simulink model "model_compatible"  (Simulink 8.7)
(part 8 of 11)

  _CN_29344008_220000_CN_25306938_220000 : powerlib/Elements/Distributed Parameters Line  Phases=3  Frequency=50  Resistance=[0.01273 0.3864]  Inductance="[0.9337e-3  4.1264e-3]"  Capacitance=[12.74e-9 7.751e-9]  Length=40.0884  x1=[8.73114913702011e-11 380000 380000;314.159265358979 314.159265358979 314.159265358979;-0.177670123217348 0.415246442777429 -1.15554988401747]  x2=[1.26090477118469e-09 381852.398472139 381852.398472139;314.159265358979 314.159265358979 314.159265358979;-1.41941675517191 0.415007521738739 -1.15578880505616]  x3=[1.07663708898761e-11 1405.24743813465 1405.24743813466;314.159265358979 314.159265358979 314.159265358979;-2.70558821102223 0.316110507002444 -1.25468581979246]  x4=[8.62234243168895e-12 1405.96374414071 1405.9637441407;314.159265358979 314.159265358979 314.159265358979;0.245769282942371 0.405640215255436 -1.16515611153945]  x5=0.000565541566995742  V1=ones(3,3)  V2=ones(3,3)  I1=ones(3,3)  I2=ones(3,3)  nHarmo=1  Measurements=None
  _CN_29344008_220000_CN_28008024_220000 : powerlib/Elements/Distributed Parameters Line  Phases=3  Frequency=50  Resistance=[0.01273 0.3864]  Inductance="[0.9337e-3  4.1264e-3]"  Capacitance=[12.74e-9 7.751e-9]  Length=70.9833  x1=[8.73114913702011e-11 380000 380000;314.159265358979 314.159265358979 314.159265358979;-0.177670123217348 0.415246442777429 -1.15554988401747]  x2=[1.26090477118469e-09 381852.398472139 381852.398472139;314.159265358979 314.159265358979 314.159265358979;-1.41941675517191 0.415007521738739 -1.15578880505616]  x3=[1.07663708898761e-11 1405.24743813465 1405.24743813466;314.159265358979 314.159265358979 314.159265358979;-2.70558821102223 0.316110507002444 -1.25468581979246]  x4=[8.62234243168895e-12 1405.96374414071 1405.9637441407;314.159265358979 314.159265358979 314.159265358979;0.245769282942371 0.405640215255436 -1.16515611153945]  x5=0.000565541566995742  V1=ones(3,3)  V2=ones(3,3)  I1=ones(3,3)  I2=ones(3,3)  nHarmo=1  Measurements=None
  _CN_29344008_220000_CN_33017336_220000 : powerlib/Elements/Distributed Parameters Line  Phases=3  Frequency=50  Resistance=[0.01273 0.3864]  Inductance="[0.9337e-3  4.1264e-3]"  Capacitance=[12.74e-9 7.751e-9]  Length=11.7304  x1=[8.73114913702011e-11 380000 380000;314.159265358979 314.159265358979 314.159265358979;-0.177670123217348 0.415246442777429 -1.15554988401747]  x2=[1.26090477118469e-09 381852.398472139 381852.398472139;314.159265358979 314.159265358979 314.159265358979;-1.41941675517191 0.415007521738739 -1.15578880505616]  x3=[1.07663708898761e-11 1405.24743813465 1405.24743813466;314.159265358979 314.159265358979 314.159265358979;-2.70558821102223 0.316110507002444 -1.25468581979246]  x4=[8.62234243168895e-12 1405.96374414071 1405.9637441407;314.159265358979 314.159265358979 314.159265358979;0.245769282942371 0.405640215255436 -1.16515611153945]  x5=0.000565541566995742  V1=ones(3,3)  V2=ones(3,3)  I1=ones(3,3)  I2=ones(3,3)  nHarmo=1  Measurements=None
  _CN_29472852_220000_CN_114319248_220000 : powerlib/Elements/Distributed Parameters Line  Phases=3  Frequency=50  Resistance=[0.01273 0.3864]  Inductance="[0.9337e-3  4.1264e-3]"  Capacitance=[12.74e-9 7.751e-9]  Length=21.4615  x1=[8.73114913702011e-11 380000 380000;314.159265358979 314.159265358979 314.159265358979;-0.177670123217348 0.415246442777429 -1.15554988401747]  x2=[1.26090477118469e-09 381852.398472139 381852.398472139;314.159265358979 314.159265358979 314.159265358979;-1.41941675517191 0.415007521738739 -1.15578880505616]  x3=[1.07663708898761e-11 1405.24743813465 1405.24743813466;314.159265358979 314.159265358979 314.159265358979;-2.70558821102223 0.316110507002444 -1.25468581979246]  x4=[8.62234243168895e-12 1405.96374414071 1405.9637441407;314.159265358979 314.159265358979 314.159265358979;0.245769282942371 0.405640215255436 -1.16515611153945]  x5=0.000565541566995742  V1=ones(3,3)  V2=ones(3,3)  I1=ones(3,3)  I2=ones(3,3)  nHarmo=1  Measurements=None
  _CN_29472852_220000_CN_37764852_220000 : powerlib/Elements/Distributed Parameters Line  Phases=3  Frequency=50  Resistance=[0.01273 0.3864]  Inductance="[0.9337e-3  4.1264e-3]"  Capacitance=[12.74e-9 7.751e-9]  Length=46.7716  x1=[8.73114913702011e-11 380000 380000;314.159265358979 314.159265358979 314.159265358979;-0.177670123217348 0.415246442777429 -1.15554988401747]  x2=[1.26090477118469e-09 381852.398472139 381852.398472139;314.159265358979 314.159265358979 314.159265358979;-1.41941675517191 0.415007521738739 -1.15578880505616]  x3=[1.07663708898761e-11 1405.24743813465 1405.24743813466;314.159265358979 314.159265358979 314.159265358979;-2.70558821102223 0.316110507002444 -1.25468581979246]  x4=[8.62234243168895e-12 1405.96374414071 1405.9637441407;314.159265358979 314.159265358979 314.159265358979;0.245769282942371 0.405640215255436 -1.16515611153945]  x5=0.000565541566995742  V1=ones(3,3)  V2=ones(3,3)  I1=ones(3,3)  I2=ones(3,3)  nHarmo=1  Measurements=None
  _CN_29713902_380000_CN218161891 : powerlib/Elements/Distributed Parameters Line  Phases=3  Frequency=50  Resistance=[0.01273 0.3864]  Inductance="[0.9337e-3  4.1264e-3]"  Capacitance=[12.74e-9 7.751e-9]  Length=8.2062  x1=[8.73114913702011e-11 380000 380000;314.159265358979 314.159265358979 314.159265358979;-0.177670123217348 0.415246442777429 -1.15554988401747]  x2=[1.26090477118469e-09 381852.398472139 381852.398472139;314.159265358979 314.159265358979 314.159265358979;-1.41941675517191 0.415007521738739 -1.15578880505616]  x3=[1.07663708898761e-11 1405.24743813465 1405.24743813466;314.159265358979 314.159265358979 314.159265358979;-2.70558821102223 0.316110507002444 -1.25468581979246]  x4=[8.62234243168895e-12 1405.96374414071 1405.9637441407;314.159265358979 314.159265358979 314.159265358979;0.245769282942371 0.405640215255436 -1.16515611153945]  x5=0.000565541566995742  V1=ones(3,3)  V2=ones(3,3)  I1=ones(3,3)  I2=ones(3,3)  nHarmo=1  Measurements=None
  _CN_30132758_380000_CN_43163132_380000 : powerlib/Elements/Distributed Parameters Line  Phases=3  Frequency=50  Resistance=[0.01273 0.3864]  Inductance="[0.9337e-3  4.1264e-3]"  Capacitance=[12.74e-9 7.751e-9]  Length=12.8168  x1=[8.73114913702011e-11 380000 380000;314.159265358979 314.159265358979 314.159265358979;-0.177670123217348 0.415246442777429 -1.15554988401747]  x2=[1.26090477118469e-09 381852.398472139 381852.398472139;314.159265358979 314.159265358979 314.159265358979;-1.41941675517191 0.415007521738739 -1.15578880505616]  x3=[1.07663708898761e-11 1405.24743813465 1405.24743813466;314.159265358979 314.159265358979 314.159265358979;-2.70558821102223 0.316110507002444 -1.25468581979246]  x4=[8.62234243168895e-12 1405.96374414071 1405.9637441407;314.159265358979 314.159265358979 314.159265358979;0.245769282942371 0.405640215255436 -1.16515611153945]  x5=0.000565541566995742  V1=ones(3,3)  V2=ones(3,3)  I1=ones(3,3)  I2=ones(3,3)  nHarmo=1  Measurements=None
  _CN_30164703_380000_CN58421134 : powerlib/Elements/Distributed Parameters Line  Phases=3  Frequency=50  Resistance=[0.01273 0.3864]  Inductance="[0.9337e-3  4.1264e-3]"  Capacitance=[12.74e-9 7.751e-9]  Length=15.2286  x1=[8.73114913702011e-11 380000 380000;314.159265358979 314.159265358979 314.159265358979;-0.177670123217348 0.415246442777429 -1.15554988401747]  x2=[1.26090477118469e-09 381852.398472139 381852.398472139;314.159265358979 314.159265358979 314.159265358979;-1.41941675517191 0.415007521738739 -1.15578880505616]  x3=[1.07663708898761e-11 1405.24743813465 1405.24743813466;314.159265358979 314.159265358979 314.159265358979;-2.70558821102223 0.316110507002444 -1.25468581979246]  x4=[8.62234243168895e-12 1405.96374414071 1405.9637441407;314.159265358979 314.159265358979 314.159265358979;0.245769282942371 0.405640215255436 -1.16515611153945]  x5=0.000565541566995742  V1=ones(3,3)  V2=ones(3,3)  I1=ones(3,3)  I2=ones(3,3)  nHarmo=1  Measurements=None
  _CN_30613895_220000_CN_31019937_220000 : powerlib/Elements/Distributed Parameters Line  Phases=3  Frequency=50  Resistance=[0.01273 0.3864]  Inductance="[0.9337e-3  4.1264e-3]"  Capacitance=[12.74e-9 7.751e-9]  Length=89.562  x1=[8.73114913702011e-11 380000 380000;314.159265358979 314.159265358979 314.159265358979;-0.177670123217348 0.415246442777429 -1.15554988401747]  x2=[1.26090477118469e-09 381852.398472139 381852.398472139;314.159265358979 314.159265358979 314.159265358979;-1.41941675517191 0.415007521738739 -1.15578880505616]  x3=[1.07663708898761e-11 1405.24743813465 1405.24743813466;314.159265358979 314.159265358979 314.159265358979;-2.70558821102223 0.316110507002444 -1.25468581979246]  x4=[8.62234243168895e-12 1405.96374414071 1405.9637441407;314.159265358979 314.159265358979 314.159265358979;0.245769282942371 0.405640215255436 -1.16515611153945]  x5=0.000565541566995742  V1=ones(3,3)  V2=ones(3,3)  I1=ones(3,3)  I2=ones(3,3)  nHarmo=1  Measurements=None
  _CN_30613895_380000_CN_24652261_380000 : powerlib/Elements/Distributed Parameters Line  Phases=3  Frequency=50  Resistance=[0.01273 0.3864]  Inductance="[0.9337e-3  4.1264e-3]"  Capacitance=[12.74e-9 7.751e-9]  Length=77.7493  x1=[8.73114913702011e-11 380000 380000;314.159265358979 314.159265358979 314.159265358979;-0.177670123217348 0.415246442777429 -1.15554988401747]  x2=[1.26090477118469e-09 381852.398472139 381852.398472139;314.159265358979 314.159265358979 314.159265358979;-1.41941675517191 0.415007521738739 -1.15578880505616]  x3=[1.07663708898761e-11 1405.24743813465 1405.24743813466;314.159265358979 314.159265358979 314.159265358979;-2.70558821102223 0.316110507002444 -1.25468581979246]  x4=[8.62234243168895e-12 1405.96374414071 1405.9637441407;314.159265358979 314.159265358979 314.159265358979;0.245769282942371 0.405640215255436 -1.16515611153945]  x5=0.000565541566995742  V1=ones(3,3)  V2=ones(3,3)  I1=ones(3,3)  I2=ones(3,3)  nHarmo=1  Measurements=None
  _CN_30613895_380000_CN_53378027_380000 : powerlib/Elements/Distributed Parameters Line  Phases=3  Frequency=50  Resistance=[0.01273 0.3864]  Inductance="[0.9337e-3  4.1264e-3]"  Capacitance=[12.74e-9 7.751e-9]  Length=52.887  x1=[8.73114913702011e-11 380000 380000;314.159265358979 314.159265358979 314.159265358979;-0.177670123217348 0.415246442777429 -1.15554988401747]  x2=[1.26090477118469e-09 381852.398472139 381852.398472139;314.159265358979 314.159265358979 314.159265358979;-1.41941675517191 0.415007521738739 -1.15578880505616]  x3=[1.07663708898761e-11 1405.24743813465 1405.24743813466;314.159265358979 314.159265358979 314.159265358979;-2.70558821102223 0.316110507002444 -1.25468581979246]  x4=[8.62234243168895e-12 1405.96374414071 1405.9637441407;314.159265358979 314.159265358979 314.159265358979;0.245769282942371 0.405640215255436 -1.16515611153945]  x5=0.000565541566995742  V1=ones(3,3)  V2=ones(3,3)  I1=ones(3,3)  I2=ones(3,3)  nHarmo=1  Measurements=None
  _CN_30622610_220000_CN55015415 : powerlib/Elements/Distributed Parameters Line  Phases=3  Frequency=50  Resistance=[0.01273 0.3864]  Inductance="[0.9337e-3  4.1264e-3]"  Capacitance=[12.74e-9 7.751e-9]  Length=30.8042  x1=[8.73114913702011e-11 380000 380000;314.159265358979 314.159265358979 314.159265358979;-0.177670123217348 0.415246442777429 -1.15554988401747]  x2=[1.26090477118469e-09 381852.398472139 381852.398472139;314.159265358979 314.159265358979 314.159265358979;-1.41941675517191 0.415007521738739 -1.15578880505616]  x3=[1.07663708898761e-11 1405.24743813465 1405.24743813466;314.159265358979 314.159265358979 314.159265358979;-2.70558821102223 0.316110507002444 -1.25468581979246]  x4=[8.62234243168895e-12 1405.96374414071 1405.9637441407;314.159265358979 314.159265358979 314.159265358979;0.245769282942371 0.405640215255436 -1.16515611153945]  x5=0.000565541566995742  V1=ones(3,3)  V2=ones(3,3)  I1=ones(3,3)  I2=ones(3,3)  nHarmo=1  Measurements=None
  _CN_31019937_380000_CN_85523877_380000 : powerlib/Elements/Distributed Parameters Line  Phases=3  Frequency=50  Resistance=[0.01273 0.3864]  Inductance="[0.9337e-3  4.1264e-3]"  Capacitance=[12.74e-9 7.751e-9]  Length=0.24167  x1=[8.73114913702011e-11 380000 380000;314.159265358979 314.159265358979 314.159265358979;-0.177670123217348 0.415246442777429 -1.15554988401747]  x2=[1.26090477118469e-09 381852.398472139 381852.398472139;314.159265358979 314.159265358979 314.159265358979;-1.41941675517191 0.415007521738739 -1.15578880505616]  x3=[1.07663708898761e-11 1405.24743813465 1405.24743813466;314.159265358979 314.159265358979 314.159265358979;-2.70558821102223 0.316110507002444 -1.25468581979246]  x4=[8.62234243168895e-12 1405.96374414071 1405.9637441407;314.159265358979 314.159265358979 314.159265358979;0.245769282942371 0.405640215255436 -1.16515611153945]  x5=0.000565541566995742  V1=ones(3,3)  V2=ones(3,3)  I1=ones(3,3)  I2=ones(3,3)  nHarmo=1  Measurements=None
  _CN_31131320_380000_CN_31131325_380000 : powerlib/Elements/Distributed Parameters Line  Phases=3  Frequency=50  Resistance=[0.01273 0.3864]  Inductance="[0.9337e-3  4.1264e-3]"  Capacitance=[12.74e-9 7.751e-9]  Length=27.2208  x1=[8.73114913702011e-11 380000 380000;314.159265358979 314.159265358979 314.159265358979;-0.177670123217348 0.415246442777429 -1.15554988401747]  x2=[1.26090477118469e-09 381852.398472139 381852.398472139;314.159265358979 314.159265358979 314.159265358979;-1.41941675517191 0.415007521738739 -1.15578880505616]  x3=[1.07663708898761e-11 1405.24743813465 1405.24743813466;314.159265358979 314.159265358979 314.159265358979;-2.70558821102223 0.316110507002444 -1.25468581979246]  x4=[8.62234243168895e-12 1405.96374414071 1405.9637441407;314.159265358979 314.159265358979 314.159265358979;0.245769282942371 0.405640215255436 -1.16515611153945]  x5=0.000565541566995742  V1=ones(3,3)  V2=ones(3,3)  I1=ones(3,3)  I2=ones(3,3)  nHarmo=1  Measurements=None
  _CN_31367937_220000_CN_87653464_220000 : powerlib/Elements/Distributed Parameters Line  Phases=3  Frequency=50  Resistance=[0.01273 0.3864]  Inductance="[0.9337e-3  4.1264e-3]"  Capacitance=[12.74e-9 7.751e-9]  Length=100  x1=[8.73114913702011e-11 380000 380000;314.159265358979 314.159265358979 314.159265358979;-0.177670123217348 0.415246442777429 -1.15554988401747]  x2=[1.26090477118469e-09 381852.398472139 381852.398472139;314.159265358979 314.159265358979 314.159265358979;-1.41941675517191 0.415007521738739 -1.15578880505616]  x3=[1.07663708898761e-11 1405.24743813465 1405.24743813466;314.159265358979 314.159265358979 314.159265358979;-2.70558821102223 0.316110507002444 -1.25468581979246]  x4=[8.62234243168895e-12 1405.96374414071 1405.9637441407;314.159265358979 314.159265358979 314.159265358979;0.245769282942371 0.405640215255436 -1.16515611153945]  x5=0.000565541566995742  V1=ones(3,3)  V2=ones(3,3)  I1=ones(3,3)  I2=ones(3,3)  nHarmo=1  Measurements=None
  _CN_32076853_380000_CN_109582315_380000 : powerlib/Elements/Distributed Parameters Line  Phases=3  Frequency=50  Resistance=[0.01273 0.3864]  Inductance="[0.9337e-3  4.1264e-3]"  Capacitance=[12.74e-9 7.751e-9]  Length=0.34614  x1=[8.73114913702011e-11 380000 380000;314.159265358979 314.159265358979 314.159265358979;-0.177670123217348 0.415246442777429 -1.15554988401747]  x2=[1.26090477118469e-09 381852.398472139 381852.398472139;314.159265358979 314.159265358979 314.159265358979;-1.41941675517191 0.415007521738739 -1.15578880505616]  x3=[1.07663708898761e-11 1405.24743813465 1405.24743813466;314.159265358979 314.159265358979 314.159265358979;-2.70558821102223 0.316110507002444 -1.25468581979246]  x4=[8.62234243168895e-12 1405.96374414071 1405.9637441407;314.159265358979 314.159265358979 314.159265358979;0.245769282942371 0.405640215255436 -1.16515611153945]  x5=0.000565541566995742  V1=ones(3,3)  V2=ones(3,3)  I1=ones(3,3)  I2=ones(3,3)  nHarmo=1  Measurements=None
  _CN_32151621_220000_CN_146962222_220000 : powerlib/Elements/Distributed Parameters Line  Phases=3  Frequency=50  Resistance=[0.01273 0.3864]  Inductance="[0.9337e-3  4.1264e-3]"  Capacitance=[12.74e-9 7.751e-9]  Length=72.3935  x1=[8.73114913702011e-11 380000 380000;314.159265358979 314.159265358979 314.159265358979;-0.177670123217348 0.415246442777429 -1.15554988401747]  x2=[1.26090477118469e-09 381852.398472139 381852.398472139;314.159265358979 314.159265358979 314.159265358979;-1.41941675517191 0.415007521738739 -1.15578880505616]  x3=[1.07663708898761e-11 1405.24743813465 1405.24743813466;314.159265358979 314.159265358979 314.159265358979;-2.70558821102223 0.316110507002444 -1.25468581979246]  x4=[8.62234243168895e-12 1405.96374414071 1405.9637441407;314.159265358979 314.159265358979 314.159265358979;0.245769282942371 0.405640215255436 -1.16515611153945]  x5=0.000565541566995742  V1=ones(3,3)  V2=ones(3,3)  I1=ones(3,3)  I2=ones(3,3)  nHarmo=1  Measurements=None
  _CN_32151621_220000_CN_152261133_220000 : powerlib/Elements/Distributed Parameters Line  Phases=3  Frequency=50  Resistance=[0.01273 0.3864]  Inductance="[0.9337e-3  4.1264e-3]"  Capacitance=[12.74e-9 7.751e-9]  Length=30.7373  x1=[8.73114913702011e-11 380000 380000;314.159265358979 314.159265358979 314.159265358979;-0.177670123217348 0.415246442777429 -1.15554988401747]  x2=[1.26090477118469e-09 381852.398472139 381852.398472139;314.159265358979 314.159265358979 314.159265358979;-1.41941675517191 0.415007521738739 -1.15578880505616]  x3=[1.07663708898761e-11 1405.24743813465 1405.24743813466;314.159265358979 314.159265358979 314.159265358979;-2.70558821102223 0.316110507002444 -1.25468581979246]  x4=[8.62234243168895e-12 1405.96374414071 1405.9637441407;314.159265358979 314.159265358979 314.159265358979;0.245769282942371 0.405640215255436 -1.16515611153945]  x5=0.000565541566995742  V1=ones(3,3)  V2=ones(3,3)  I1=ones(3,3)  I2=ones(3,3)  nHarmo=1  Measurements=None
  _CN_32151621_220000_CN_39011884_220000 : powerlib/Elements/Distributed Parameters Line  Phases=3  Frequency=50  Resistance=[0.01273 0.3864]  Inductance="[0.9337e-3  4.1264e-3]"  Capacitance=[12.74e-9 7.751e-9]  Length=33.2187  x1=[8.73114913702011e-11 380000 380000;314.159265358979 314.159265358979 314.159265358979;-0.177670123217348 0.415246442777429 -1.15554988401747]  x2=[1.26090477118469e-09 381852.398472139 381852.398472139;314.159265358979 314.159265358979 314.159265358979;-1.41941675517191 0.415007521738739 -1.15578880505616]  x3=[1.07663708898761e-11 1405.24743813465 1405.24743813466;314.159265358979 314.159265358979 314.159265358979;-2.70558821102223 0.316110507002444 -1.25468581979246]  x4=[8.62234243168895e-12 1405.96374414071 1405.9637441407;314.159265358979 314.159265358979 314.159265358979;0.245769282942371 0.405640215255436 -1.16515611153945]  x5=0.000565541566995742  V1=ones(3,3)  V2=ones(3,3)  I1=ones(3,3)  I2=ones(3,3)  nHarmo=1  Measurements=None
  _CN_32318130_220000_CN_29389718_220000 : powerlib/Elements/Distributed Parameters Line  Phases=3  Frequency=50  Resistance=[0.01273 0.3864]  Inductance="[0.9337e-3  4.1264e-3]"  Capacitance=[12.74e-9 7.751e-9]  Length=12.1297  x1=[8.73114913702011e-11 380000 380000;314.159265358979 314.159265358979 314.159265358979;-0.177670123217348 0.415246442777429 -1.15554988401747]  x2=[1.26090477118469e-09 381852.398472139 381852.398472139;314.159265358979 314.159265358979 314.159265358979;-1.41941675517191 0.415007521738739 -1.15578880505616]  x3=[1.07663708898761e-11 1405.24743813465 1405.24743813466;314.159265358979 314.159265358979 314.159265358979;-2.70558821102223 0.316110507002444 -1.25468581979246]  x4=[8.62234243168895e-12 1405.96374414071 1405.9637441407;314.159265358979 314.159265358979 314.159265358979;0.245769282942371 0.405640215255436 -1.16515611153945]  x5=0.000565541566995742  V1=ones(3,3)  V2=ones(3,3)  I1=ones(3,3)  I2=ones(3,3)  nHarmo=1  Measurements=None
  _CN_32318130_220000_CN_32062544_220000 : powerlib/Elements/Distributed Parameters Line  Phases=3  Frequency=50  Resistance=[0.01273 0.3864]  Inductance="[0.9337e-3  4.1264e-3]"  Capacitance=[12.74e-9 7.751e-9]  Length=70.4994  x1=[8.73114913702011e-11 380000 380000;314.159265358979 314.159265358979 314.159265358979;-0.177670123217348 0.415246442777429 -1.15554988401747]  x2=[1.26090477118469e-09 381852.398472139 381852.398472139;314.159265358979 314.159265358979 314.159265358979;-1.41941675517191 0.415007521738739 -1.15578880505616]  x3=[1.07663708898761e-11 1405.24743813465 1405.24743813466;314.159265358979 314.159265358979 314.159265358979;-2.70558821102223 0.316110507002444 -1.25468581979246]  x4=[8.62234243168895e-12 1405.96374414071 1405.9637441407;314.159265358979 314.159265358979 314.159265358979;0.245769282942371 0.405640215255436 -1.16515611153945]  x5=0.000565541566995742  V1=ones(3,3)  V2=ones(3,3)  I1=ones(3,3)  I2=ones(3,3)  nHarmo=1  Measurements=None
  _CN_32725957_220000_CN_32725958_220000 : powerlib/Elements/Distributed Parameters Line  Phases=3  Frequency=50  Resistance=[0.01273 0.3864]  Inductance="[0.9337e-3  4.1264e-3]"  Capacitance=[12.74e-9 7.751e-9]  Length=4.0892  x1=[8.73114913702011e-11 380000 380000;314.159265358979 314.159265358979 314.159265358979;-0.177670123217348 0.415246442777429 -1.15554988401747]  x2=[1.26090477118469e-09 381852.398472139 381852.398472139;314.159265358979 314.159265358979 314.159265358979;-1.41941675517191 0.415007521738739 -1.15578880505616]  x3=[1.07663708898761e-11 1405.24743813465 1405.24743813466;314.159265358979 314.159265358979 314.159265358979;-2.70558821102223 0.316110507002444 -1.25468581979246]  x4=[8.62234243168895e-12 1405.96374414071 1405.9637441407;314.159265358979 314.159265358979 314.159265358979;0.245769282942371 0.405640215255436 -1.16515611153945]  x5=0.000565541566995742  V1=ones(3,3)  V2=ones(3,3)  I1=ones(3,3)  I2=ones(3,3)  nHarmo=1  Measurements=None
  _CN_33042984_220000_CN_160093341_220000 : powerlib/Elements/Distributed Parameters Line  Phases=3  Frequency=50  Resistance=[0.01273 0.3864]  Inductance="[0.9337e-3  4.1264e-3]"  Capacitance=[12.74e-9 7.751e-9]  Length=107.68  x1=[8.73114913702011e-11 380000 380000;314.159265358979 314.159265358979 314.159265358979;-0.177670123217348 0.415246442777429 -1.15554988401747]  x2=[1.26090477118469e-09 381852.398472139 381852.398472139;314.159265358979 314.159265358979 314.159265358979;-1.41941675517191 0.415007521738739 -1.15578880505616]  x3=[1.07663708898761e-11 1405.24743813465 1405.24743813466;314.159265358979 314.159265358979 314.159265358979;-2.70558821102223 0.316110507002444 -1.25468581979246]  x4=[8.62234243168895e-12 1405.96374414071 1405.9637441407;314.159265358979 314.159265358979 314.159265358979;0.245769282942371 0.405640215255436 -1.16515611153945]  x5=0.000565541566995742  V1=ones(3,3)  V2=ones(3,3)  I1=ones(3,3)  I2=ones(3,3)  nHarmo=1  Measurements=None
  _CN_33042984_220000_CN_30109913_220000 : powerlib/Elements/Distributed Parameters Line  Phases=3  Frequency=50  Resistance=[0.01273 0.3864]  Inductance="[0.9337e-3  4.1264e-3]"  Capacitance=[12.74e-9 7.751e-9]  Length=79.2206  x1=[8.73114913702011e-11 380000 380000;314.159265358979 314.159265358979 314.159265358979;-0.177670123217348 0.415246442777429 -1.15554988401747]  x2=[1.26090477118469e-09 381852.398472139 381852.398472139;314.159265358979 314.159265358979 314.159265358979;-1.41941675517191 0.415007521738739 -1.15578880505616]  x3=[1.07663708898761e-11 1405.24743813465 1405.24743813466;314.159265358979 314.159265358979 314.159265358979;-2.70558821102223 0.316110507002444 -1.25468581979246]  x4=[8.62234243168895e-12 1405.96374414071 1405.9637441407;314.159265358979 314.159265358979 314.159265358979;0.245769282942371 0.405640215255436 -1.16515611153945]  x5=0.000565541566995742  V1=ones(3,3)  V2=ones(3,3)  I1=ones(3,3)  I2=ones(3,3)  nHarmo=1  Measurements=None
  _CN_33042984_220000_CN_43072656_220000 : powerlib/Elements/Distributed Parameters Line  Phases=3  Frequency=50  Resistance=[0.01273 0.3864]  Inductance="[0.9337e-3  4.1264e-3]"  Capacitance=[12.74e-9 7.751e-9]  Length=148.7412  x1=[8.73114913702011e-11 380000 380000;314.159265358979 314.159265358979 314.159265358979;-0.177670123217348 0.415246442777429 -1.15554988401747]  x2=[1.26090477118469e-09 381852.398472139 381852.398472139;314.159265358979 314.159265358979 314.159265358979;-1.41941675517191 0.415007521738739 -1.15578880505616]  x3=[1.07663708898761e-11 1405.24743813465 1405.24743813466;314.159265358979 314.159265358979 314.159265358979;-2.70558821102223 0.316110507002444 -1.25468581979246]  x4=[8.62234243168895e-12 1405.96374414071 1405.9637441407;314.159265358979 314.159265358979 314.159265358979;0.245769282942371 0.405640215255436 -1.16515611153945]  x5=0.000565541566995742  V1=ones(3,3)  V2=ones(3,3)  I1=ones(3,3)  I2=ones(3,3)  nHarmo=1  Measurements=None
  _CN_33411203_220000_CN_114319248_220000 : powerlib/Elements/Distributed Parameters Line  Phases=3  Frequency=50  Resistance=[0.01273 0.3864]  Inductance="[0.9337e-3  4.1264e-3]"  Capacitance=[12.74e-9 7.751e-9]  Length=100.8638  x1=[8.73114913702011e-11 380000 380000;314.159265358979 314.159265358979 314.159265358979;-0.177670123217348 0.415246442777429 -1.15554988401747]  x2=[1.26090477118469e-09 381852.398472139 381852.398472139;314.159265358979 314.159265358979 314.159265358979;-1.41941675517191 0.415007521738739 -1.15578880505616]  x3=[1.07663708898761e-11 1405.24743813465 1405.24743813466;314.159265358979 314.159265358979 314.159265358979;-2.70558821102223 0.316110507002444 -1.25468581979246]  x4=[8.62234243168895e-12 1405.96374414071 1405.9637441407;314.159265358979 314.159265358979 314.159265358979;0.245769282942371 0.405640215255436 -1.16515611153945]  x5=0.000565541566995742  V1=ones(3,3)  V2=ones(3,3)  I1=ones(3,3)  I2=ones(3,3)  nHarmo=1  Measurements=None
  _CN_33411203_220000_CN_37764852_220000 : powerlib/Elements/Distributed Parameters Line  Phases=3  Frequency=50  Resistance=[0.01273 0.3864]  Inductance="[0.9337e-3  4.1264e-3]"  Capacitance=[12.74e-9 7.751e-9]  Length=34.2315  x1=[8.73114913702011e-11 380000 380000;314.159265358979 314.159265358979 314.159265358979;-0.177670123217348 0.415246442777429 -1.15554988401747]  x2=[1.26090477118469e-09 381852.398472139 381852.398472139;314.159265358979 314.159265358979 314.159265358979;-1.41941675517191 0.415007521738739 -1.15578880505616]  x3=[1.07663708898761e-11 1405.24743813465 1405.24743813466;314.159265358979 314.159265358979 314.159265358979;-2.70558821102223 0.316110507002444 -1.25468581979246]  x4=[8.62234243168895e-12 1405.96374414071 1405.9637441407;314.159265358979 314.159265358979 314.159265358979;0.245769282942371 0.405640215255436 -1.16515611153945]  x5=0.000565541566995742  V1=ones(3,3)  V2=ones(3,3)  I1=ones(3,3)  I2=ones(3,3)  nHarmo=1  Measurements=None
  _CN_33411203_380000_CN_24604789_380000 : powerlib/Elements/Distributed Parameters Line  Phases=3  Frequency=50  Resistance=[0.01273 0.3864]  Inductance="[0.9337e-3  4.1264e-3]"  Capacitance=[12.74e-9 7.751e-9]  Length=143.1283  x1=[8.73114913702011e-11 380000 380000;314.159265358979 314.159265358979 314.159265358979;-0.177670123217348 0.415246442777429 -1.15554988401747]  x2=[1.26090477118469e-09 381852.398472139 381852.398472139;314.159265358979 314.159265358979 314.159265358979;-1.41941675517191 0.415007521738739 -1.15578880505616]  x3=[1.07663708898761e-11 1405.24743813465 1405.24743813466;314.159265358979 314.159265358979 314.159265358979;-2.70558821102223 0.316110507002444 -1.25468581979246]  x4=[8.62234243168895e-12 1405.96374414071 1405.9637441407;314.159265358979 314.159265358979 314.159265358979;0.245769282942371 0.405640215255436 -1.16515611153945]  x5=0.000565541566995742  V1=ones(3,3)  V2=ones(3,3)  I1=ones(3,3)  I2=ones(3,3)  nHarmo=1  Measurements=None
  _CN_33411203_380000_CN_27739871_380000 : powerlib/Elements/Distributed Parameters Line  Phases=3  Frequency=50  Resistance=[0.01273 0.3864]  Inductance="[0.9337e-3  4.1264e-3]"  Capacitance=[12.74e-9 7.751e-9]  Length=129.6976  x1=[8.73114913702011e-11 380000 380000;314.159265358979 314.159265358979 314.159265358979;-0.177670123217348 0.415246442777429 -1.15554988401747]  x2=[1.26090477118469e-09 381852.398472139 381852.398472139;314.159265358979 314.159265358979 314.159265358979;-1.41941675517191 0.415007521738739 -1.15578880505616]  x3=[1.07663708898761e-11 1405.24743813465 1405.24743813466;314.159265358979 314.159265358979 314.159265358979;-2.70558821102223 0.316110507002444 -1.25468581979246]  x4=[8.62234243168895e-12 1405.96374414071 1405.9637441407;314.159265358979 314.159265358979 314.159265358979;0.245769282942371 0.405640215255436 -1.16515611153945]  x5=0.000565541566995742  V1=ones(3,3)  V2=ones(3,3)  I1=ones(3,3)  I2=ones(3,3)  nHarmo=1  Measurements=None
  _CN_35818137_220000_CN_35818522_220000 : powerlib/Elements/Distributed Parameters Line  Phases=3  Frequency=50  Resistance=[0.01273 0.3864]  Inductance="[0.9337e-3  4.1264e-3]"  Capacitance=[12.74e-9 7.751e-9]  Length=1.6839  x1=[8.73114913702011e-11 380000 380000;314.159265358979 314.159265358979 314.159265358979;-0.177670123217348 0.415246442777429 -1.15554988401747]  x2=[1.26090477118469e-09 381852.398472139 381852.398472139;314.159265358979 314.159265358979 314.159265358979;-1.41941675517191 0.415007521738739 -1.15578880505616]  x3=[1.07663708898761e-11 1405.24743813465 1405.24743813466;314.159265358979 314.159265358979 314.159265358979;-2.70558821102223 0.316110507002444 -1.25468581979246]  x4=[8.62234243168895e-12 1405.96374414071 1405.9637441407;314.159265358979 314.159265358979 314.159265358979;0.245769282942371 0.405640215255436 -1.16515611153945]  x5=0.000565541566995742  V1=ones(3,3)  V2=ones(3,3)  I1=ones(3,3)  I2=ones(3,3)  nHarmo=1  Measurements=None
  _CN_35833442_220000_CN125808869 : powerlib/Elements/Distributed Parameters Line  Phases=3  Frequency=50  Resistance=[0.01273 0.3864]  Inductance="[0.9337e-3  4.1264e-3]"  Capacitance=[12.74e-9 7.751e-9]  Length=0.69479  x1=[8.73114913702011e-11 380000 380000;314.159265358979 314.159265358979 314.159265358979;-0.177670123217348 0.415246442777429 -1.15554988401747]  x2=[1.26090477118469e-09 381852.398472139 381852.398472139;314.159265358979 314.159265358979 314.159265358979;-1.41941675517191 0.415007521738739 -1.15578880505616]  x3=[1.07663708898761e-11 1405.24743813465 1405.24743813466;314.159265358979 314.159265358979 314.159265358979;-2.70558821102223 0.316110507002444 -1.25468581979246]  x4=[8.62234243168895e-12 1405.96374414071 1405.9637441407;314.159265358979 314.159265358979 314.159265358979;0.245769282942371 0.405640215255436 -1.16515611153945]  x5=0.000565541566995742  V1=ones(3,3)  V2=ones(3,3)  I1=ones(3,3)  I2=ones(3,3)  nHarmo=1  Measurements=None
  _CN_35833592_220000_CN_35833442_220000 : powerlib/Elements/Distributed Parameters Line  Phases=3  Frequency=50  Resistance=[0.01273 0.3864]  Inductance="[0.9337e-3  4.1264e-3]"  Capacitance=[12.74e-9 7.751e-9]  Length=2.6796  x1=[8.73114913702011e-11 380000 380000;314.159265358979 314.159265358979 314.159265358979;-0.177670123217348 0.415246442777429 -1.15554988401747]  x2=[1.26090477118469e-09 381852.398472139 381852.398472139;314.159265358979 314.159265358979 314.159265358979;-1.41941675517191 0.415007521738739 -1.15578880505616]  x3=[1.07663708898761e-11 1405.24743813465 1405.24743813466;314.159265358979 314.159265358979 314.159265358979;-2.70558821102223 0.316110507002444 -1.25468581979246]  x4=[8.62234243168895e-12 1405.96374414071 1405.9637441407;314.159265358979 314.159265358979 314.159265358979;0.245769282942371 0.405640215255436 -1.16515611153945]  x5=0.000565541566995742  V1=ones(3,3)  V2=ones(3,3)  I1=ones(3,3)  I2=ones(3,3)  nHarmo=1  Measurements=None
  _CN_39690368_220000_CN_32062544_220000 : powerlib/Elements/Distributed Parameters Line  Phases=3  Frequency=50  Resistance=[0.01273 0.3864]  Inductance="[0.9337e-3  4.1264e-3]"  Capacitance=[12.74e-9 7.751e-9]  Length=1.5793  x1=[8.73114913702011e-11 380000 380000;314.159265358979 314.159265358979 314.159265358979;-0.177670123217348 0.415246442777429 -1.15554988401747]  x2=[1.26090477118469e-09 381852.398472139 381852.398472139;314.159265358979 314.159265358979 314.159265358979;-1.41941675517191 0.415007521738739 -1.15578880505616]  x3=[1.07663708898761e-11 1405.24743813465 1405.24743813466;314.159265358979 314.159265358979 314.159265358979;-2.70558821102223 0.316110507002444 -1.25468581979246]  x4=[8.62234243168895e-12 1405.96374414071 1405.9637441407;314.159265358979 314.159265358979 314.159265358979;0.245769282942371 0.405640215255436 -1.16515611153945]  x5=0.000565541566995742  V1=ones(3,3)  V2=ones(3,3)  I1=ones(3,3)  I2=ones(3,3)  nHarmo=1  Measurements=None
  _CN_41334805_220000_CN_143903369_220000 : powerlib/Elements/Distributed Parameters Line  Phases=3  Frequency=50  Resistance=[0.01273 0.3864]  Inductance="[0.9337e-3  4.1264e-3]"  Capacitance=[12.74e-9 7.751e-9]  Length=114.5956  x1=[8.73114913702011e-11 380000 380000;314.159265358979 314.159265358979 314.159265358979;-0.177670123217348 0.415246442777429 -1.15554988401747]  x2=[1.26090477118469e-09 381852.398472139 381852.398472139;314.159265358979 314.159265358979 314.159265358979;-1.41941675517191 0.415007521738739 -1.15578880505616]  x3=[1.07663708898761e-11 1405.24743813465 1405.24743813466;314.159265358979 314.159265358979 314.159265358979;-2.70558821102223 0.316110507002444 -1.25468581979246]  x4=[8.62234243168895e-12 1405.96374414071 1405.9637441407;314.159265358979 314.159265358979 314.159265358979;0.245769282942371 0.405640215255436 -1.16515611153945]  x5=0.000565541566995742  V1=ones(3,3)  V2=ones(3,3)  I1=ones(3,3)  I2=ones(3,3)  nHarmo=1  Measurements=None
  _CN_41334805_220000_CN_152973139_220000 : powerlib/Elements/Distributed Parameters Line  Phases=3  Frequency=50  Resistance=[0.01273 0.3864]  Inductance="[0.9337e-3  4.1264e-3]"  Capacitance=[12.74e-9 7.751e-9]  Length=109.9639  x1=[8.73114913702011e-11 380000 380000;314.159265358979 314.159265358979 314.159265358979;-0.177670123217348 0.415246442777429 -1.15554988401747]  x2=[1.26090477118469e-09 381852.398472139 381852.398472139;314.159265358979 314.159265358979 314.159265358979;-1.41941675517191 0.415007521738739 -1.15578880505616]  x3=[1.07663708898761e-11 1405.24743813465 1405.24743813466;314.159265358979 314.159265358979 314.159265358979;-2.70558821102223 0.316110507002444 -1.25468581979246]  x4=[8.62234243168895e-12 1405.96374414071 1405.9637441407;314.159265358979 314.159265358979 314.159265358979;0.245769282942371 0.405640215255436 -1.16515611153945]  x5=0.000565541566995742  V1=ones(3,3)  V2=ones(3,3)  I1=ones(3,3)  I2=ones(3,3)  nHarmo=1  Measurements=None
  _CN_41334805_220000_CN_207248812_220000 : powerlib/Elements/Distributed Parameters Line  Phases=3  Frequency=50  Resistance=[0.01273 0.3864]  Inductance="[0.9337e-3  4.1264e-3]"  Capacitance=[12.74e-9 7.751e-9]  Length=93.2926  x1=[8.73114913702011e-11 380000 380000;314.159265358979 314.159265358979 314.159265358979;-0.177670123217348 0.415246442777429 -1.15554988401747]  x2=[1.26090477118469e-09 381852.398472139 381852.398472139;314.159265358979 314.159265358979 314.159265358979;-1.41941675517191 0.415007521738739 -1.15578880505616]  x3=[1.07663708898761e-11 1405.24743813465 1405.24743813466;314.159265358979 314.159265358979 314.159265358979;-2.70558821102223 0.316110507002444 -1.25468581979246]  x4=[8.62234243168895e-12 1405.96374414071 1405.9637441407;314.159265358979 314.159265358979 314.159265358979;0.245769282942371 0.405640215255436 -1.16515611153945]  x5=0.000565541566995742  V1=ones(3,3)  V2=ones(3,3)  I1=ones(3,3)  I2=ones(3,3)  nHarmo=1  Measurements=None
  _CN_41334805_220000_CN_23414063_220000 : powerlib/Elements/Distributed Parameters Line  Phases=3  Frequency=50  Resistance=[0.01273 0.3864]  Inductance="[0.9337e-3  4.1264e-3]"  Capacitance=[12.74e-9 7.751e-9]  Length=53.7382  x1=[8.73114913702011e-11 380000 380000;314.159265358979 314.159265358979 314.159265358979;-0.177670123217348 0.415246442777429 -1.15554988401747]  x2=[1.26090477118469e-09 381852.398472139 381852.398472139;314.159265358979 314.159265358979 314.159265358979;-1.41941675517191 0.415007521738739 -1.15578880505616]  x3=[1.07663708898761e-11 1405.24743813465 1405.24743813466;314.159265358979 314.159265358979 314.159265358979;-2.70558821102223 0.316110507002444 -1.25468581979246]  x4=[8.62234243168895e-12 1405.96374414071 1405.9637441407;314.159265358979 314.159265358979 314.159265358979;0.245769282942371 0.405640215255436 -1.16515611153945]  x5=0.000565541566995742  V1=ones(3,3)  V2=ones(3,3)  I1=ones(3,3)  I2=ones(3,3)  nHarmo=1  Measurements=None
  _CN_41334805_220000_CN_25557397_220000 : powerlib/Elements/Distributed Parameters Line  Phases=3  Frequency=50  Resistance=[0.01273 0.3864]  Inductance="[0.9337e-3  4.1264e-3]"  Capacitance=[12.74e-9 7.751e-9]  Length=20.269  x1=[8.73114913702011e-11 380000 380000;314.159265358979 314.159265358979 314.159265358979;-0.177670123217348 0.415246442777429 -1.15554988401747]  x2=[1.26090477118469e-09 381852.398472139 381852.398472139;314.159265358979 314.159265358979 314.159265358979;-1.41941675517191 0.415007521738739 -1.15578880505616]  x3=[1.07663708898761e-11 1405.24743813465 1405.24743813466;314.159265358979 314.159265358979 314.159265358979;-2.70558821102223 0.316110507002444 -1.25468581979246]  x4=[8.62234243168895e-12 1405.96374414071 1405.9637441407;314.159265358979 314.159265358979 314.159265358979;0.245769282942371 0.405640215255436 -1.16515611153945]  x5=0.000565541566995742  V1=ones(3,3)  V2=ones(3,3)  I1=ones(3,3)  I2=ones(3,3)  nHarmo=1  Measurements=None
  _CN_41334805_220000_CN_25786404_220000 : powerlib/Elements/Distributed Parameters Line  Phases=3  Frequency=50  Resistance=[0.01273 0.3864]  Inductance="[0.9337e-3  4.1264e-3]"  Capacitance=[12.74e-9 7.751e-9]  Length=22.5776  x1=[8.73114913702011e-11 380000 380000;314.159265358979 314.159265358979 314.159265358979;-0.177670123217348 0.415246442777429 -1.15554988401747]  x2=[1.26090477118469e-09 381852.398472139 381852.398472139;314.159265358979 314.159265358979 314.159265358979;-1.41941675517191 0.415007521738739 -1.15578880505616]  x3=[1.07663708898761e-11 1405.24743813465 1405.24743813466;314.159265358979 314.159265358979 314.159265358979;-2.70558821102223 0.316110507002444 -1.25468581979246]  x4=[8.62234243168895e-12 1405.96374414071 1405.9637441407;314.159265358979 314.159265358979 314.159265358979;0.245769282942371 0.405640215255436 -1.16515611153945]  x5=0.000565541566995742  V1=ones(3,3)  V2=ones(3,3)  I1=ones(3,3)  I2=ones(3,3)  nHarmo=1  Measurements=None
  _CN_41334805_220000_CN_43688805_220000 : powerlib/Elements/Distributed Parameters Line  Phases=3  Frequency=50  Resistance=[0.01273 0.3864]  Inductance="[0.9337e-3  4.1264e-3]"  Capacitance=[12.74e-9 7.751e-9]  Length=42.9643  x1=[8.73114913702011e-11 380000 380000;314.159265358979 314.159265358979 314.159265358979;-0.177670123217348 0.415246442777429 -1.15554988401747]  x2=[1.26090477118469e-09 381852.398472139 381852.398472139;314.159265358979 314.159265358979 314.159265358979;-1.41941675517191 0.415007521738739 -1.15578880505616]  x3=[1.07663708898761e-11 1405.24743813465 1405.24743813466;314.159265358979 314.159265358979 314.159265358979;-2.70558821102223 0.316110507002444 -1.25468581979246]  x4=[8.62234243168895e-12 1405.96374414071 1405.9637441407;314.159265358979 314.159265358979 314.159265358979;0.245769282942371 0.405640215255436 -1.16515611153945]  x5=0.000565541566995742  V1=ones(3,3)  V2=ones(3,3)  I1=ones(3,3)  I2=ones(3,3)  nHarmo=1  Measurements=None
  _CN_42410916_220000_CN145861680 : powerlib/Elements/Distributed Parameters Line  Phases=3  Frequency=50  Resistance=[0.01273 0.3864]  Inductance="[0.9337e-3  4.1264e-3]"  Capacitance=[12.74e-9 7.751e-9]  Length=1.0748  x1=[8.73114913702011e-11 380000 380000;314.159265358979 314.159265358979 314.159265358979;-0.177670123217348 0.415246442777429 -1.15554988401747]  x2=[1.26090477118469e-09 381852.398472139 381852.398472139;314.159265358979 314.159265358979 314.159265358979;-1.41941675517191 0.415007521738739 -1.15578880505616]  x3=[1.07663708898761e-11 1405.24743813465 1405.24743813466;314.159265358979 314.159265358979 314.159265358979;-2.70558821102223 0.316110507002444 -1.25468581979246]  x4=[8.62234243168895e-12 1405.96374414071 1405.9637441407;314.159265358979 314.159265358979 314.159265358979;0.245769282942371 0.405640215255436 -1.16515611153945]  x5=0.000565541566995742  V1=ones(3,3)  V2=ones(3,3)  I1=ones(3,3)  I2=ones(3,3)  nHarmo=1  Measurements=None
  _CN_42410916_220000_CN_42411962_220000 : powerlib/Elements/Distributed Parameters Line  Phases=3  Frequency=50  Resistance=[0.01273 0.3864]  Inductance="[0.9337e-3  4.1264e-3]"  Capacitance=[12.74e-9 7.751e-9]  Length=0.70686  x1=[8.73114913702011e-11 380000 380000;314.159265358979 314.159265358979 314.159265358979;-0.177670123217348 0.415246442777429 -1.15554988401747]  x2=[1.26090477118469e-09 381852.398472139 381852.398472139;314.159265358979 314.159265358979 314.159265358979;-1.41941675517191 0.415007521738739 -1.15578880505616]  x3=[1.07663708898761e-11 1405.24743813465 1405.24743813466;314.159265358979 314.159265358979 314.159265358979;-2.70558821102223 0.316110507002444 -1.25468581979246]  x4=[8.62234243168895e-12 1405.96374414071 1405.9637441407;314.159265358979 314.159265358979 314.159265358979;0.245769282942371 0.405640215255436 -1.16515611153945]  x5=0.000565541566995742  V1=ones(3,3)  V2=ones(3,3)  I1=ones(3,3)  I2=ones(3,3)  nHarmo=1  Measurements=None
  _CN_42411962_220000_CN145861680 : powerlib/Elements/Distributed Parameters Line  Phases=3  Frequency=50  Resistance=[0.01273 0.3864]  Inductance="[0.9337e-3  4.1264e-3]"  Capacitance=[12.74e-9 7.751e-9]  Length=0.1006  x1=[8.73114913702011e-11 380000 380000;314.159265358979 314.159265358979 314.159265358979;-0.177670123217348 0.415246442777429 -1.15554988401747]  x2=[1.26090477118469e-09 381852.398472139 381852.398472139;314.159265358979 314.159265358979 314.159265358979;-1.41941675517191 0.415007521738739 -1.15578880505616]  x3=[1.07663708898761e-11 1405.24743813465 1405.24743813466;314.159265358979 314.159265358979 314.159265358979;-2.70558821102223 0.316110507002444 -1.25468581979246]  x4=[8.62234243168895e-12 1405.96374414071 1405.9637441407;314.159265358979 314.159265358979 314.159265358979;0.245769282942371 0.405640215255436 -1.16515611153945]  x5=0.000565541566995742  V1=ones(3,3)  V2=ones(3,3)  I1=ones(3,3)  I2=ones(3,3)  nHarmo=1  Measurements=None
  _CN_42488855_380000_CN_112695048_380000 : powerlib/Elements/Distributed Parameters Line  Phases=3  Frequency=50  Resistance=[0.01273 0.3864]  Inductance="[0.9337e-3  4.1264e-3]"  Capacitance=[12.74e-9 7.751e-9]  Length=6.9786  x1=[8.73114913702011e-11 380000 380000;314.159265358979 314.159265358979 314.159265358979;-0.177670123217348 0.415246442777429 -1.15554988401747]  x2=[1.26090477118469e-09 381852.398472139 381852.398472139;314.159265358979 314.159265358979 314.159265358979;-1.41941675517191 0.415007521738739 -1.15578880505616]  x3=[1.07663708898761e-11 1405.24743813465 1405.24743813466;314.159265358979 314.159265358979 314.159265358979;-2.70558821102223 0.316110507002444 -1.25468581979246]  x4=[8.62234243168895e-12 1405.96374414071 1405.9637441407;314.159265358979 314.159265358979 314.159265358979;0.245769282942371 0.405640215255436 -1.16515611153945]  x5=0.000565541566995742  V1=ones(3,3)  V2=ones(3,3)  I1=ones(3,3)  I2=ones(3,3)  nHarmo=1  Measurements=None
  _CN_42488855_380000_CN_22964137_380000 : powerlib/Elements/Distributed Parameters Line  Phases=3  Frequency=50  Resistance=[0.01273 0.3864]  Inductance="[0.9337e-3  4.1264e-3]"  Capacitance=[12.74e-9 7.751e-9]  Length=86.9099  x1=[8.73114913702011e-11 380000 380000;314.159265358979 314.159265358979 314.159265358979;-0.177670123217348 0.415246442777429 -1.15554988401747]  x2=[1.26090477118469e-09 381852.398472139 381852.398472139;314.159265358979 314.159265358979 314.159265358979;-1.41941675517191 0.415007521738739 -1.15578880505616]  x3=[1.07663708898761e-11 1405.24743813465 1405.24743813466;314.159265358979 314.159265358979 314.159265358979;-2.70558821102223 0.316110507002444 -1.25468581979246]  x4=[8.62234243168895e-12 1405.96374414071 1405.9637441407;314.159265358979 314.159265358979 314.159265358979;0.245769282942371 0.405640215255436 -1.16515611153945]  x5=0.000565541566995742  V1=ones(3,3)  V2=ones(3,3)  I1=ones(3,3)  I2=ones(3,3)  nHarmo=1  Measurements=None
  _CN_42488855_380000_CN_32472806_380000 : powerlib/Elements/Distributed Parameters Line  Phases=3  Frequency=50  Resistance=[0.01273 0.3864]  Inductance="[0.9337e-3  4.1264e-3]"  Capacitance=[12.74e-9 7.751e-9]  Length=111.3469  x1=[8.73114913702011e-11 380000 380000;314.159265358979 314.159265358979 314.159265358979;-0.177670123217348 0.415246442777429 -1.15554988401747]  x2=[1.26090477118469e-09 381852.398472139 381852.398472139;314.159265358979 314.159265358979 314.159265358979;-1.41941675517191 0.415007521738739 -1.15578880505616]  x3=[1.07663708898761e-11 1405.24743813465 1405.24743813466;314.159265358979 314.159265358979 314.159265358979;-2.70558821102223 0.316110507002444 -1.25468581979246]  x4=[8.62234243168895e-12 1405.96374414071 1405.9637441407;314.159265358979 314.159265358979 314.159265358979;0.245769282942371 0.405640215255436 -1.16515611153945]  x5=0.000565541566995742  V1=ones(3,3)  V2=ones(3,3)  I1=ones(3,3)  I2=ones(3,3)  nHarmo=1  Measurements=None
  _CN_42488855_380000_CN_35763480_380000 : powerlib/Elements/Distributed Parameters Line  Phases=3  Frequency=50  Resistance=[0.01273 0.3864]  Inductance="[0.9337e-3  4.1264e-3]"  Capacitance=[12.74e-9 7.751e-9]  Length=99.4674  x1=[8.73114913702011e-11 380000 380000;314.159265358979 314.159265358979 314.159265358979;-0.177670123217348 0.415246442777429 -1.15554988401747]  x2=[1.26090477118469e-09 381852.398472139 381852.398472139;314.159265358979 314.159265358979 314.159265358979;-1.41941675517191 0.415007521738739 -1.15578880505616]  x3=[1.07663708898761e-11 1405.24743813465 1405.24743813466;314.159265358979 314.159265358979 314.159265358979;-2.70558821102223 0.316110507002444 -1.25468581979246]  x4=[8.62234243168895e-12 1405.96374414071 1405.9637441407;314.159265358979 314.159265358979 314.159265358979;0.245769282942371 0.405640215255436 -1.16515611153945]  x5=0.000565541566995742  V1=ones(3,3)  V2=ones(3,3)  I1=ones(3,3)  I2=ones(3,3)  nHarmo=1  Measurements=None
  _CN_42488855_380000_CN_42488850_380000 : powerlib/Elements/Distributed Parameters Line  Phases=3  Frequency=50  Resistance=[0.01273 0.3864]  Inductance="[0.9337e-3  4.1264e-3]"  Capacitance=[12.74e-9 7.751e-9]  Length=2.2106  x1=[8.73114913702011e-11 380000 380000;314.159265358979 314.159265358979 314.159265358979;-0.177670123217348 0.415246442777429 -1.15554988401747]  x2=[1.26090477118469e-09 381852.398472139 381852.398472139;314.159265358979 314.159265358979 314.159265358979;-1.41941675517191 0.415007521738739 -1.15578880505616]  x3=[1.07663708898761e-11 1405.24743813465 1405.24743813466;314.159265358979 314.159265358979 314.159265358979;-2.70558821102223 0.316110507002444 -1.25468581979246]  x4=[8.62234243168895e-12 1405.96374414071 1405.9637441407;314.159265358979 314.159265358979 314.159265358979;0.245769282942371 0.405640215255436 -1.16515611153945]  x5=0.000565541566995742  V1=ones(3,3)  V2=ones(3,3)  I1=ones(3,3)  I2=ones(3,3)  nHarmo=1  Measurements=None
  _CN_42488855_380000_CN_42809973_380000 : powerlib/Elements/Distributed Parameters Line  Phases=3  Frequency=50  Resistance=[0.01273 0.3864]  Inductance="[0.9337e-3  4.1264e-3]"  Capacitance=[12.74e-9 7.751e-9]  Length=46.214  x1=[8.73114913702011e-11 380000 380000;314.159265358979 314.159265358979 314.159265358979;-0.177670123217348 0.415246442777429 -1.15554988401747]  x2=[1.26090477118469e-09 381852.398472139 381852.398472139;314.159265358979 314.159265358979 314.159265358979;-1.41941675517191 0.415007521738739 -1.15578880505616]  x3=[1.07663708898761e-11 1405.24743813465 1405.24743813466;314.159265358979 314.159265358979 314.159265358979;-2.70558821102223 0.316110507002444 -1.25468581979246]  x4=[8.62234243168895e-12 1405.96374414071 1405.9637441407;314.159265358979 314.159265358979 314.159265358979;0.245769282942371 0.405640215255436 -1.16515611153945]  x5=0.000565541566995742  V1=ones(3,3)  V2=ones(3,3)  I1=ones(3,3)  I2=ones(3,3)  nHarmo=1  Measurements=None
  _CN_42681484_380000_CN_24413992_380000 : powerlib/Elements/Distributed Parameters Line  Phases=3  Frequency=50  Resistance=[0.01273 0.3864]  Inductance="[0.9337e-3  4.1264e-3]"  Capacitance=[12.74e-9 7.751e-9]  Length=47.1732  x1=[8.73114913702011e-11 380000 380000;314.159265358979 314.159265358979 314.159265358979;-0.177670123217348 0.415246442777429 -1.15554988401747]  x2=[1.26090477118469e-09 381852.398472139 381852.398472139;314.159265358979 314.159265358979 314.159265358979;-1.41941675517191 0.415007521738739 -1.15578880505616]  x3=[1.07663708898761e-11 1405.24743813465 1405.24743813466;314.159265358979 314.159265358979 314.159265358979;-2.70558821102223 0.316110507002444 -1.25468581979246]  x4=[8.62234243168895e-12 1405.96374414071 1405.9637441407;314.159265358979 314.159265358979 314.159265358979;0.245769282942371 0.405640215255436 -1.16515611153945]  x5=0.000565541566995742  V1=ones(3,3)  V2=ones(3,3)  I1=ones(3,3)  I2=ones(3,3)  nHarmo=1  Measurements=None
  _CN_42681484_380000_CN_274630377_380000 : powerlib/Elements/Distributed Parameters Line  Phases=3  Frequency=50  Resistance=[0.01273 0.3864]  Inductance="[0.9337e-3  4.1264e-3]"  Capacitance=[12.74e-9 7.751e-9]  Length=45.3031  x1=[8.73114913702011e-11 380000 380000;314.159265358979 314.159265358979 314.159265358979;-0.177670123217348 0.415246442777429 -1.15554988401747]  x2=[1.26090477118469e-09 381852.398472139 381852.398472139;314.159265358979 314.159265358979 314.159265358979;-1.41941675517191 0.415007521738739 -1.15578880505616]  x3=[1.07663708898761e-11 1405.24743813465 1405.24743813466;314.159265358979 314.159265358979 314.159265358979;-2.70558821102223 0.316110507002444 -1.25468581979246]  x4=[8.62234243168895e-12 1405.96374414071 1405.9637441407;314.159265358979 314.159265358979 314.159265358979;0.245769282942371 0.405640215255436 -1.16515611153945]  x5=0.000565541566995742  V1=ones(3,3)  V2=ones(3,3)  I1=ones(3,3)  I2=ones(3,3)  nHarmo=1  Measurements=None
  _CN_43163132_380000_CN185569568 : powerlib/Elements/Distributed Parameters Line  Phases=3  Frequency=50  Resistance=[0.01273 0.3864]  Inductance="[0.9337e-3  4.1264e-3]"  Capacitance=[12.74e-9 7.751e-9]  Length=2.1561  x1=[8.73114913702011e-11 380000 380000;314.159265358979 314.159265358979 314.159265358979;-0.177670123217348 0.415246442777429 -1.15554988401747]  x2=[1.26090477118469e-09 381852.398472139 381852.398472139;314.159265358979 314.159265358979 314.159265358979;-1.41941675517191 0.415007521738739 -1.15578880505616]  x3=[1.07663708898761e-11 1405.24743813465 1405.24743813466;314.159265358979 314.159265358979 314.159265358979;-2.70558821102223 0.316110507002444 -1.25468581979246]  x4=[8.62234243168895e-12 1405.96374414071 1405.9637441407;314.159265358979 314.159265358979 314.159265358979;0.245769282942371 0.405640215255436 -1.16515611153945]  x5=0.000565541566995742  V1=ones(3,3)  V2=ones(3,3)  I1=ones(3,3)  I2=ones(3,3)  nHarmo=1  Measurements=None
  _CN_46766896_220000_CN_90807341_220000 : powerlib/Elements/Distributed Parameters Line  Phases=3  Frequency=50  Resistance=[0.01273 0.3864]  Inductance="[0.9337e-3  4.1264e-3]"  Capacitance=[12.74e-9 7.751e-9]  Length=0.24571  x1=[8.73114913702011e-11 380000 380000;314.159265358979 314.159265358979 314.159265358979;-0.177670123217348 0.415246442777429 -1.15554988401747]  x2=[1.26090477118469e-09 381852.398472139 381852.398472139;314.159265358979 314.159265358979 314.159265358979;-1.41941675517191 0.415007521738739 -1.15578880505616]  x3=[1.07663708898761e-11 1405.24743813465 1405.24743813466;314.159265358979 314.159265358979 314.159265358979;-2.70558821102223 0.316110507002444 -1.25468581979246]  x4=[8.62234243168895e-12 1405.96374414071 1405.9637441407;314.159265358979 314.159265358979 314.159265358979;0.245769282942371 0.405640215255436 -1.16515611153945]  x5=0.000565541566995742  V1=ones(3,3)  V2=ones(3,3)  I1=ones(3,3)  I2=ones(3,3)  nHarmo=1  Measurements=None
  _CN_54359256_220000_CN30425117 : powerlib/Elements/Distributed Parameters Line  Phases=3  Frequency=50  Resistance=[0.01273 0.3864]  Inductance="[0.9337e-3  4.1264e-3]"  Capacitance=[12.74e-9 7.751e-9]  Length=9.0385  x1=[8.73114913702011e-11 380000 380000;314.159265358979 314.159265358979 314.159265358979;-0.177670123217348 0.415246442777429 -1.15554988401747]  x2=[1.26090477118469e-09 381852.398472139 381852.398472139;314.159265358979 314.159265358979 314.159265358979;-1.41941675517191 0.415007521738739 -1.15578880505616]  x3=[1.07663708898761e-11 1405.24743813465 1405.24743813466;314.159265358979 314.159265358979 314.159265358979;-2.70558821102223 0.316110507002444 -1.25468581979246]  x4=[8.62234243168895e-12 1405.96374414071 1405.9637441407;314.159265358979 314.159265358979 314.159265358979;0.245769282942371 0.405640215255436 -1.16515611153945]  x5=0.000565541566995742  V1=ones(3,3)  V2=ones(3,3)  I1=ones(3,3)  I2=ones(3,3)  nHarmo=1  Measurements=None
  _CN_54359256_220000_CN_100812630_220000 : powerlib/Elements/Distributed Parameters Line  Phases=3  Frequency=50  Resistance=[0.01273 0.3864]  Inductance="[0.9337e-3  4.1264e-3]"  Capacitance=[12.74e-9 7.751e-9]  Length=9.0478  x1=[8.73114913702011e-11 380000 380000;314.159265358979 314.159265358979 314.159265358979;-0.177670123217348 0.415246442777429 -1.15554988401747]  x2=[1.26090477118469e-09 381852.398472139 381852.398472139;314.159265358979 314.159265358979 314.159265358979;-1.41941675517191 0.415007521738739 -1.15578880505616]  x3=[1.07663708898761e-11 1405.24743813465 1405.24743813466;314.159265358979 314.159265358979 314.159265358979;-2.70558821102223 0.316110507002444 -1.25468581979246]  x4=[8.62234243168895e-12 1405.96374414071 1405.9637441407;314.159265358979 314.159265358979 314.159265358979;0.245769282942371 0.405640215255436 -1.16515611153945]  x5=0.000565541566995742  V1=ones(3,3)  V2=ones(3,3)  I1=ones(3,3)  I2=ones(3,3)  nHarmo=1  Measurements=None
  _CN_54359256_380000_CN115145869 : powerlib/Elements/Distributed Parameters Line  Phases=3  Frequency=50  Resistance=[0.01273 0.3864]  Inductance="[0.9337e-3  4.1264e-3]"  Capacitance=[12.74e-9 7.751e-9]  Length=35.9283  x1=[8.73114913702011e-11 380000 380000;314.159265358979 314.159265358979 314.159265358979;-0.177670123217348 0.415246442777429 -1.15554988401747]  x2=[1.26090477118469e-09 381852.398472139 381852.398472139;314.159265358979 314.159265358979 314.159265358979;-1.41941675517191 0.415007521738739 -1.15578880505616]  x3=[1.07663708898761e-11 1405.24743813465 1405.24743813466;314.159265358979 314.159265358979 314.159265358979;-2.70558821102223 0.316110507002444 -1.25468581979246]  x4=[8.62234243168895e-12 1405.96374414071 1405.9637441407;314.159265358979 314.159265358979 314.159265358979;0.245769282942371 0.405640215255436 -1.16515611153945]  x5=0.000565541566995742  V1=ones(3,3)  V2=ones(3,3)  I1=ones(3,3)  I2=ones(3,3)  nHarmo=1  Measurements=None
  _CN_59026005_380000_CN_157807291_380000 : powerlib/Elements/Distributed Parameters Line  Phases=3  Frequency=50  Resistance=[0.01273 0.3864]  Inductance="[0.9337e-3  4.1264e-3]"  Capacitance=[12.74e-9 7.751e-9]  Length=90.2072  x1=[8.73114913702011e-11 380000 380000;314.159265358979 314.159265358979 314.159265358979;-0.177670123217348 0.415246442777429 -1.15554988401747]  x2=[1.26090477118469e-09 381852.398472139 381852.398472139;314.159265358979 314.159265358979 314.159265358979;-1.41941675517191 0.415007521738739 -1.15578880505616]  x3=[1.07663708898761e-11 1405.24743813465 1405.24743813466;314.159265358979 314.159265358979 314.159265358979;-2.70558821102223 0.316110507002444 -1.25468581979246]  x4=[8.62234243168895e-12 1405.96374414071 1405.9637441407;314.159265358979 314.159265358979 314.159265358979;0.245769282942371 0.405640215255436 -1.16515611153945]  x5=0.000565541566995742  V1=ones(3,3)  V2=ones(3,3)  I1=ones(3,3)  I2=ones(3,3)  nHarmo=1  Measurements=None
  _CN_59925390_380000_CN_113546939_380000 : powerlib/Elements/Distributed Parameters Line  Phases=3  Frequency=50  Resistance=[0.01273 0.3864]  Inductance="[0.9337e-3  4.1264e-3]"  Capacitance=[12.74e-9 7.751e-9]  Length=23.5758  x1=[8.73114913702011e-11 380000 380000;314.159265358979 314.159265358979 314.159265358979;-0.177670123217348 0.415246442777429 -1.15554988401747]  x2=[1.26090477118469e-09 381852.398472139 381852.398472139;314.159265358979 314.159265358979 314.159265358979;-1.41941675517191 0.415007521738739 -1.15578880505616]  x3=[1.07663708898761e-11 1405.24743813465 1405.24743813466;314.159265358979 314.159265358979 314.159265358979;-2.70558821102223 0.316110507002444 -1.25468581979246]  x4=[8.62234243168895e-12 1405.96374414071 1405.9637441407;314.159265358979 314.159265358979 314.159265358979;0.245769282942371 0.405640215255436 -1.16515611153945]  x5=0.000565541566995742  V1=ones(3,3)  V2=ones(3,3)  I1=ones(3,3)  I2=ones(3,3)  nHarmo=1  Measurements=None
  _CN_60032354_220000_CN55015415 : powerlib/Elements/Distributed Parameters Line  Phases=3  Frequency=50  Resistance=[0.01273 0.3864]  Inductance="[0.9337e-3  4.1264e-3]"  Capacitance=[12.74e-9 7.751e-9]  Length=0.32568  x1=[8.73114913702011e-11 380000 380000;314.159265358979 314.159265358979 314.159265358979;-0.177670123217348 0.415246442777429 -1.15554988401747]  x2=[1.26090477118469e-09 381852.398472139 381852.398472139;314.159265358979 314.159265358979 314.159265358979;-1.41941675517191 0.415007521738739 -1.15578880505616]  x3=[1.07663708898761e-11 1405.24743813465 1405.24743813466;314.159265358979 314.159265358979 314.159265358979;-2.70558821102223 0.316110507002444 -1.25468581979246]  x4=[8.62234243168895e-12 1405.96374414071 1405.9637441407;314.159265358979 314.159265358979 314.159265358979;0.245769282942371 0.405640215255436 -1.16515611153945]  x5=0.000565541566995742  V1=ones(3,3)  V2=ones(3,3)  I1=ones(3,3)  I2=ones(3,3)  nHarmo=1  Measurements=None
  _CN_61918154_380000_CN49339874 : powerlib/Elements/Distributed Parameters Line  Phases=3  Frequency=50  Resistance=[0.01273 0.3864]  Inductance="[0.9337e-3  4.1264e-3]"  Capacitance=[12.74e-9 7.751e-9]  Length=1.4703  x1=[8.73114913702011e-11 380000 380000;314.159265358979 314.159265358979 314.159265358979;-0.177670123217348 0.415246442777429 -1.15554988401747]  x2=[1.26090477118469e-09 381852.398472139 381852.398472139;314.159265358979 314.159265358979 314.159265358979;-1.41941675517191 0.415007521738739 -1.15578880505616]  x3=[1.07663708898761e-11 1405.24743813465 1405.24743813466;314.159265358979 314.159265358979 314.159265358979;-2.70558821102223 0.316110507002444 -1.25468581979246]  x4=[8.62234243168895e-12 1405.96374414071 1405.9637441407;314.159265358979 314.159265358979 314.159265358979;0.245769282942371 0.405640215255436 -1.16515611153945]  x5=0.000565541566995742  V1=ones(3,3)  V2=ones(3,3)  I1=ones(3,3)  I2=ones(3,3)  nHarmo=1  Measurements=None
  _CN_63114179_380000_CN_35763480_380000 : powerlib/Elements/Distributed Parameters Line  Phases=3  Frequency=50  Resistance=[0.01273 0.3864]  Inductance="[0.9337e-3  4.1264e-3]"  Capacitance=[12.74e-9 7.751e-9]  Length=28.0497  x1=[8.73114913702011e-11 380000 380000;314.159265358979 314.159265358979 314.159265358979;-0.177670123217348 0.415246442777429 -1.15554988401747]  x2=[1.26090477118469e-09 381852.398472139 381852.398472139;314.159265358979 314.159265358979 314.159265358979;-1.41941675517191 0.415007521738739 -1.15578880505616]  x3=[1.07663708898761e-11 1405.24743813465 1405.24743813466;314.159265358979 314.159265358979 314.159265358979;-2.70558821102223 0.316110507002444 -1.25468581979246]  x4=[8.62234243168895e-12 1405.96374414071 1405.9637441407;314.159265358979 314.159265358979 314.159265358979;0.245769282942371 0.405640215255436 -1.16515611153945]  x5=0.000565541566995742  V1=ones(3,3)  V2=ones(3,3)  I1=ones(3,3)  I2=ones(3,3)  nHarmo=1  Measurements=None
  _CN_66038431_220000_CN131986820 : powerlib/Elements/Distributed Parameters Line  Phases=3  Frequency=50  Resistance=[0.01273 0.3864]  Inductance="[0.9337e-3  4.1264e-3]"  Capacitance=[12.74e-9 7.751e-9]  Length=60.8249  x1=[8.73114913702011e-11 380000 380000;314.159265358979 314.159265358979 314.159265358979;-0.177670123217348 0.415246442777429 -1.15554988401747]  x2=[1.26090477118469e-09 381852.398472139 381852.398472139;314.159265358979 314.159265358979 314.159265358979;-1.41941675517191 0.415007521738739 -1.15578880505616]  x3=[1.07663708898761e-11 1405.24743813465 1405.24743813466;314.159265358979 314.159265358979 314.159265358979;-2.70558821102223 0.316110507002444 -1.25468581979246]  x4=[8.62234243168895e-12 1405.96374414071 1405.9637441407;314.159265358979 314.159265358979 314.159265358979;0.245769282942371 0.405640215255436 -1.16515611153945]  x5=0.000565541566995742  V1=ones(3,3)  V2=ones(3,3)  I1=ones(3,3)  I2=ones(3,3)  nHarmo=1  Measurements=None
  _CN_66038431_220000_CN_113546939_220000 : powerlib/Elements/Distributed Parameters Line  Phases=3  Frequency=50  Resistance=[0.01273 0.3864]  Inductance="[0.9337e-3  4.1264e-3]"  Capacitance=[12.74e-9 7.751e-9]  Length=43.3852  x1=[8.73114913702011e-11 380000 380000;314.159265358979 314.159265358979 314.159265358979;-0.177670123217348 0.415246442777429 -1.15554988401747]  x2=[1.26090477118469e-09 381852.398472139 381852.398472139;314.159265358979 314.159265358979 314.159265358979;-1.41941675517191 0.415007521738739 -1.15578880505616]  x3=[1.07663708898761e-11 1405.24743813465 1405.24743813466;314.159265358979 314.159265358979 314.159265358979;-2.70558821102223 0.316110507002444 -1.25468581979246]  x4=[8.62234243168895e-12 1405.96374414071 1405.9637441407;314.159265358979 314.159265358979 314.159265358979;0.245769282942371 0.405640215255436 -1.16515611153945]  x5=0.000565541566995742  V1=ones(3,3)  V2=ones(3,3)  I1=ones(3,3)  I2=ones(3,3)  nHarmo=1  Measurements=None
  _CN_66038431_220000_CN_24667346_220000 : powerlib/Elements/Distributed Parameters Line  Phases=3  Frequency=50  Resistance=[0.01273 0.3864]  Inductance="[0.9337e-3  4.1264e-3]"  Capacitance=[12.74e-9 7.751e-9]  Length=67.0965  x1=[8.73114913702011e-11 380000 380000;314.159265358979 314.159265358979 314.159265358979;-0.177670123217348 0.415246442777429 -1.15554988401747]  x2=[1.26090477118469e-09 381852.398472139 381852.398472139;314.159265358979 314.159265358979 314.159265358979;-1.41941675517191 0.415007521738739 -1.15578880505616]  x3=[1.07663708898761e-11 1405.24743813465 1405.24743813466;314.159265358979 314.159265358979 314.159265358979;-2.70558821102223 0.316110507002444 -1.25468581979246]  x4=[8.62234243168895e-12 1405.96374414071 1405.9637441407;314.159265358979 314.159265358979 314.159265358979;0.245769282942371 0.405640215255436 -1.16515611153945]  x5=0.000565541566995742  V1=ones(3,3)  V2=ones(3,3)  I1=ones(3,3)  I2=ones(3,3)  nHarmo=1  Measurements=None
  _CN_66038431_220000_CN_28452784_220000 : powerlib/Elements/Distributed Parameters Line  Phases=3  Frequency=50  Resistance=[0.01273 0.3864]  Inductance="[0.9337e-3  4.1264e-3]"  Capacitance=[12.74e-9 7.751e-9]  Length=20.5572  x1=[8.73114913702011e-11 380000 380000;314.159265358979 314.159265358979 314.159265358979;-0.177670123217348 0.415246442777429 -1.15554988401747]  x2=[1.26090477118469e-09 381852.398472139 381852.398472139;314.159265358979 314.159265358979 314.159265358979;-1.41941675517191 0.415007521738739 -1.15578880505616]  x3=[1.07663708898761e-11 1405.24743813465 1405.24743813466;314.159265358979 314.159265358979 314.159265358979;-2.70558821102223 0.316110507002444 -1.25468581979246]  x4=[8.62234243168895e-12 1405.96374414071 1405.9637441407;314.159265358979 314.159265358979 314.159265358979;0.245769282942371 0.405640215255436 -1.16515611153945]  x5=0.000565541566995742  V1=ones(3,3)  V2=ones(3,3)  I1=ones(3,3)  I2=ones(3,3)  nHarmo=1  Measurements=None
  _CN_68532663_220000_CN252655527 : powerlib/Elements/Distributed Parameters Line  Phases=3  Frequency=50  Resistance=[0.01273 0.3864]  Inductance="[0.9337e-3  4.1264e-3]"  Capacitance=[12.74e-9 7.751e-9]  Length=0.11054  x1=[8.73114913702011e-11 380000 380000;314.159265358979 314.159265358979 314.159265358979;-0.177670123217348 0.415246442777429 -1.15554988401747]  x2=[1.26090477118469e-09 381852.398472139 381852.398472139;314.159265358979 314.159265358979 314.159265358979;-1.41941675517191 0.415007521738739 -1.15578880505616]  x3=[1.07663708898761e-11 1405.24743813465 1405.24743813466;314.159265358979 314.159265358979 314.159265358979;-2.70558821102223 0.316110507002444 -1.25468581979246]  x4=[8.62234243168895e-12 1405.96374414071 1405.9637441407;314.159265358979 314.159265358979 314.159265358979;0.245769282942371 0.405640215255436 -1.16515611153945]  x5=0.000565541566995742  V1=ones(3,3)  V2=ones(3,3)  I1=ones(3,3)  I2=ones(3,3)  nHarmo=1  Measurements=None
  _CN_68532663_220000_CN_24237879_220000 : powerlib/Elements/Distributed Parameters Line  Phases=3  Frequency=50  Resistance=[0.01273 0.3864]  Inductance="[0.9337e-3  4.1264e-3]"  Capacitance=[12.74e-9 7.751e-9]  Length=107.5033  x1=[8.73114913702011e-11 380000 380000;314.159265358979 314.159265358979 314.159265358979;-0.177670123217348 0.415246442777429 -1.15554988401747]  x2=[1.26090477118469e-09 381852.398472139 381852.398472139;314.159265358979 314.159265358979 314.159265358979;-1.41941675517191 0.415007521738739 -1.15578880505616]  x3=[1.07663708898761e-11 1405.24743813465 1405.24743813466;314.159265358979 314.159265358979 314.159265358979;-2.70558821102223 0.316110507002444 -1.25468581979246]  x4=[8.62234243168895e-12 1405.96374414071 1405.9637441407;314.159265358979 314.159265358979 314.159265358979;0.245769282942371 0.405640215255436 -1.16515611153945]  x5=0.000565541566995742  V1=ones(3,3)  V2=ones(3,3)  I1=ones(3,3)  I2=ones(3,3)  nHarmo=1  Measurements=None
  _CN_74893659_380000_CN_74893662_380000 : powerlib/Elements/Distributed Parameters Line  Phases=3  Frequency=50  Resistance=[0.01273 0.3864]  Inductance="[0.9337e-3  4.1264e-3]"  Capacitance=[12.74e-9 7.751e-9]  Length=5.071  x1=[8.73114913702011e-11 380000 380000;314.159265358979 314.159265358979 314.159265358979;-0.177670123217348 0.415246442777429 -1.15554988401747]  x2=[1.26090477118469e-09 381852.398472139 381852.398472139;314.159265358979 314.159265358979 314.159265358979;-1.41941675517191 0.415007521738739 -1.15578880505616]  x3=[1.07663708898761e-11 1405.24743813465 1405.24743813466;314.159265358979 314.159265358979 314.159265358979;-2.70558821102223 0.316110507002444 -1.25468581979246]  x4=[8.62234243168895e-12 1405.96374414071 1405.9637441407;314.159265358979 314.159265358979 314.159265358979;0.245769282942371 0.405640215255436 -1.16515611153945]  x5=0.000565541566995742  V1=ones(3,3)  V2=ones(3,3)  I1=ones(3,3)  I2=ones(3,3)  nHarmo=1  Measurements=None
  _CN_76185022_380000_CN26623135 : powerlib/Elements/Distributed Parameters Line  Phases=3  Frequency=50  Resistance=[0.01273 0.3864]  Inductance="[0.9337e-3  4.1264e-3]"  Capacitance=[12.74e-9 7.751e-9]  Length=9.9331  x1=[8.73114913702011e-11 380000 380000;314.159265358979 314.159265358979 314.159265358979;-0.177670123217348 0.415246442777429 -1.15554988401747]  x2=[1.26090477118469e-09 381852.398472139 381852.398472139;314.159265358979 314.159265358979 314.159265358979;-1.41941675517191 0.415007521738739 -1.15578880505616]  x3=[1.07663708898761e-11 1405.24743813465 1405.24743813466;314.159265358979 314.159265358979 314.159265358979;-2.70558821102223 0.316110507002444 -1.25468581979246]  x4=[8.62234243168895e-12 1405.96374414071 1405.9637441407;314.159265358979 314.159265358979 314.159265358979;0.245769282942371 0.405640215255436 -1.16515611153945]  x5=0.000565541566995742  V1=ones(3,3)  V2=ones(3,3)  I1=ones(3,3)  I2=ones(3,3)  nHarmo=1  Measurements=None
  _CN_77697810_380000_CN23802422 : powerlib/Elements/Distributed Parameters Line  Phases=3  Frequency=50  Resistance=[0.01273 0.3864]  Inductance="[0.9337e-3  4.1264e-3]"  Capacitance=[12.74e-9 7.751e-9]  Length=0.29708  x1=[8.73114913702011e-11 380000 380000;314.159265358979 314.159265358979 314.159265358979;-0.177670123217348 0.415246442777429 -1.15554988401747]  x2=[1.26090477118469e-09 381852.398472139 381852.398472139;314.159265358979 314.159265358979 314.159265358979;-1.41941675517191 0.415007521738739 -1.15578880505616]  x3=[1.07663708898761e-11 1405.24743813465 1405.24743813466;314.159265358979 314.159265358979 314.159265358979;-2.70558821102223 0.316110507002444 -1.25468581979246]  x4=[8.62234243168895e-12 1405.96374414071 1405.9637441407;314.159265358979 314.159265358979 314.159265358979;0.245769282942371 0.405640215255436 -1.16515611153945]  x5=0.000565541566995742  V1=ones(3,3)  V2=ones(3,3)  I1=ones(3,3)  I2=ones(3,3)  nHarmo=1  Measurements=None
  _CN_77697810_380000_CN_24976300_380000 : powerlib/Elements/Distributed Parameters Line  Phases=3  Frequency=50  Resistance=[0.01273 0.3864]  Inductance="[0.9337e-3  4.1264e-3]"  Capacitance=[12.74e-9 7.751e-9]  Length=96.0007  x1=[8.73114913702011e-11 380000 380000;314.159265358979 314.159265358979 314.159265358979;-0.177670123217348 0.415246442777429 -1.15554988401747]  x2=[1.26090477118469e-09 381852.398472139 381852.398472139;314.159265358979 314.159265358979 314.159265358979;-1.41941675517191 0.415007521738739 -1.15578880505616]  x3=[1.07663708898761e-11 1405.24743813465 1405.24743813466;314.159265358979 314.159265358979 314.159265358979;-2.70558821102223 0.316110507002444 -1.25468581979246]  x4=[8.62234243168895e-12 1405.96374414071 1405.9637441407;314.159265358979 314.159265358979 314.159265358979;0.245769282942371 0.405640215255436 -1.16515611153945]  x5=0.000565541566995742  V1=ones(3,3)  V2=ones(3,3)  I1=ones(3,3)  I2=ones(3,3)  nHarmo=1  Measurements=None
  _CN_82310607_220000_CN_90109304_220000 : powerlib/Elements/Distributed Parameters Line  Phases=3  Frequency=50  Resistance=[0.01273 0.3864]  Inductance="[0.9337e-3  4.1264e-3]"  Capacitance=[12.74e-9 7.751e-9]  Length=1.995  x1=[8.73114913702011e-11 380000 380000;314.159265358979 314.159265358979 314.159265358979;-0.177670123217348 0.415246442777429 -1.15554988401747]  x2=[1.26090477118469e-09 381852.398472139 381852.398472139;314.159265358979 314.159265358979 314.159265358979;-1.41941675517191 0.415007521738739 -1.15578880505616]  x3=[1.07663708898761e-11 1405.24743813465 1405.24743813466;314.159265358979 314.159265358979 314.159265358979;-2.70558821102223 0.316110507002444 -1.25468581979246]  x4=[8.62234243168895e-12 1405.96374414071 1405.9637441407;314.159265358979 314.159265358979 314.159265358979;0.245769282942371 0.405640215255436 -1.16515611153945]  x5=0.000565541566995742  V1=ones(3,3)  V2=ones(3,3)  I1=ones(3,3)  I2=ones(3,3)  nHarmo=1  Measurements=None
  _CN_82773910_380000_CN115145869 : powerlib/Elements/Distributed Parameters Line  Phases=3  Frequency=50  Resistance=[0.01273 0.3864]  Inductance="[0.9337e-3  4.1264e-3]"  Capacitance=[12.74e-9 7.751e-9]  Length=0.4107  x1=[8.73114913702011e-11 380000 380000;314.159265358979 314.159265358979 314.159265358979;-0.177670123217348 0.415246442777429 -1.15554988401747]  x2=[1.26090477118469e-09 381852.398472139 381852.398472139;314.159265358979 314.159265358979 314.159265358979;-1.41941675517191 0.415007521738739 -1.15578880505616]  x3=[1.07663708898761e-11 1405.24743813465 1405.24743813466;314.159265358979 314.159265358979 314.159265358979;-2.70558821102223 0.316110507002444 -1.25468581979246]  x4=[8.62234243168895e-12 1405.96374414071 1405.9637441407;314.159265358979 314.159265358979 314.159265358979;0.245769282942371 0.405640215255436 -1.16515611153945]  x5=0.000565541566995742  V1=ones(3,3)  V2=ones(3,3)  I1=ones(3,3)  I2=ones(3,3)  nHarmo=1  Measurements=None
  _CN_85523877_380000_CN_41389594_380000 : powerlib/Elements/Distributed Parameters Line  Phases=3  Frequency=50  Resistance=[0.01273 0.3864]  Inductance="[0.9337e-3  4.1264e-3]"  Capacitance=[12.74e-9 7.751e-9]  Length=24.9705  x1=[8.73114913702011e-11 380000 380000;314.159265358979 314.159265358979 314.159265358979;-0.177670123217348 0.415246442777429 -1.15554988401747]  x2=[1.26090477118469e-09 381852.398472139 381852.398472139;314.159265358979 314.159265358979 314.159265358979;-1.41941675517191 0.415007521738739 -1.15578880505616]  x3=[1.07663708898761e-11 1405.24743813465 1405.24743813466;314.159265358979 314.159265358979 314.159265358979;-2.70558821102223 0.316110507002444 -1.25468581979246]  x4=[8.62234243168895e-12 1405.96374414071 1405.9637441407;314.159265358979 314.159265358979 314.159265358979;0.245769282942371 0.405640215255436 -1.16515611153945]  x5=0.000565541566995742  V1=ones(3,3)  V2=ones(3,3)  I1=ones(3,3)  I2=ones(3,3)  nHarmo=1  Measurements=None
  _CN_87653464_220000_CN_146962222_220000 : powerlib/Elements/Distributed Parameters Line  Phases=3  Frequency=50  Resistance=[0.01273 0.3864]  Inductance="[0.9337e-3  4.1264e-3]"  Capacitance=[12.74e-9 7.751e-9]  Length=73.4581  x1=[8.73114913702011e-11 380000 380000;314.159265358979 314.159265358979 314.159265358979;-0.177670123217348 0.415246442777429 -1.15554988401747]  x2=[1.26090477118469e-09 381852.398472139 381852.398472139;314.159265358979 314.159265358979 314.159265358979;-1.41941675517191 0.415007521738739 -1.15578880505616]  x3=[1.07663708898761e-11 1405.24743813465 1405.24743813466;314.159265358979 314.159265358979 314.159265358979;-2.70558821102223 0.316110507002444 -1.25468581979246]  x4=[8.62234243168895e-12 1405.96374414071 1405.9637441407;314.159265358979 314.159265358979 314.159265358979;0.245769282942371 0.405640215255436 -1.16515611153945]  x5=0.000565541566995742  V1=ones(3,3)  V2=ones(3,3)  I1=ones(3,3)  I2=ones(3,3)  nHarmo=1  Measurements=None
  _CN_87952821_220000_CN_33148774_220000 : powerlib/Elements/Distributed Parameters Line  Phases=3  Frequency=50  Resistance=[0.01273 0.3864]  Inductance="[0.9337e-3  4.1264e-3]"  Capacitance=[12.74e-9 7.751e-9]  Length=108.9257  x1=[8.73114913702011e-11 380000 380000;314.159265358979 314.159265358979 314.159265358979;-0.177670123217348 0.415246442777429 -1.15554988401747]  x2=[1.26090477118469e-09 381852.398472139 381852.398472139;314.159265358979 314.159265358979 314.159265358979;-1.41941675517191 0.415007521738739 -1.15578880505616]  x3=[1.07663708898761e-11 1405.24743813465 1405.24743813466;314.159265358979 314.159265358979 314.159265358979;-2.70558821102223 0.316110507002444 -1.25468581979246]  x4=[8.62234243168895e-12 1405.96374414071 1405.9637441407;314.159265358979 314.159265358979 314.159265358979;0.245769282942371 0.405640215255436 -1.16515611153945]  x5=0.000565541566995742  V1=ones(3,3)  V2=ones(3,3)  I1=ones(3,3)  I2=ones(3,3)  nHarmo=1  Measurements=None
  _CN_88916034_220000_CN_202865176_220000 : powerlib/Elements/Distributed Parameters Line  Phases=3  Frequency=50  Resistance=[0.01273 0.3864]  Inductance="[0.9337e-3  4.1264e-3]"  Capacitance=[12.74e-9 7.751e-9]  Length=4.7602  x1=[8.73114913702011e-11 380000 380000;314.159265358979 314.159265358979 314.159265358979;-0.177670123217348 0.415246442777429 -1.15554988401747]  x2=[1.26090477118469e-09 381852.398472139 381852.398472139;314.159265358979 314.159265358979 314.159265358979;-1.41941675517191 0.415007521738739 -1.15578880505616]  x3=[1.07663708898761e-11 1405.24743813465 1405.24743813466;314.159265358979 314.159265358979 314.159265358979;-2.70558821102223 0.316110507002444 -1.25468581979246]  x4=[8.62234243168895e-12 1405.96374414071 1405.9637441407;314.159265358979 314.159265358979 314.159265358979;0.245769282942371 0.405640215255436 -1.16515611153945]  x5=0.000565541566995742  V1=ones(3,3)  V2=ones(3,3)  I1=ones(3,3)  I2=ones(3,3)  nHarmo=1  Measurements=None
  _CN_88916034_380000_CN_152261133_380000 : powerlib/Elements/Distributed Parameters Line  Phases=3  Frequency=50  Resistance=[0.01273 0.3864]  Inductance="[0.9337e-3  4.1264e-3]"  Capacitance=[12.74e-9 7.751e-9]  Length=231.1897  x1=[8.73114913702011e-11 380000 380000;314.159265358979 314.159265358979 314.159265358979;-0.177670123217348 0.415246442777429 -1.15554988401747]  x2=[1.26090477118469e-09 381852.398472139 381852.398472139;314.159265358979 314.159265358979 314.159265358979;-1.41941675517191 0.415007521738739 -1.15578880505616]  x3=[1.07663708898761e-11 1405.24743813465 1405.24743813466;314.159265358979 314.159265358979 314.159265358979;-2.70558821102223 0.316110507002444 -1.25468581979246]  x4=[8.62234243168895e-12 1405.96374414071 1405.9637441407;314.159265358979 314.159265358979 314.159265358979;0.245769282942371 0.405640215255436 -1.16515611153945]  x5=0.000565541566995742  V1=ones(3,3)  V2=ones(3,3)  I1=ones(3,3)  I2=ones(3,3)  nHarmo=1  Measurements=None
  _CN_88916034_380000_CN_202865177_380000 : powerlib/Elements/Distributed Parameters Line  Phases=3  Frequency=50  Resistance=[0.01273 0.3864]  Inductance="[0.9337e-3  4.1264e-3]"  Capacitance=[12.74e-9 7.751e-9]  Length=10.4694  x1=[8.73114913702011e-11 380000 380000;314.159265358979 314.159265358979 314.159265358979;-0.177670123217348 0.415246442777429 -1.15554988401747]  x2=[1.26090477118469e-09 381852.398472139 381852.398472139;314.159265358979 314.159265358979 314.159265358979;-1.41941675517191 0.415007521738739 -1.15578880505616]  x3=[1.07663708898761e-11 1405.24743813465 1405.24743813466;314.159265358979 314.159265358979 314.159265358979;-2.70558821102223 0.316110507002444 -1.25468581979246]  x4=[8.62234243168895e-12 1405.96374414071 1405.9637441407;314.159265358979 314.159265358979 314.159265358979;0.245769282942371 0.405640215255436 -1.16515611153945]  x5=0.000565541566995742  V1=ones(3,3)  V2=ones(3,3)  I1=ones(3,3)  I2=ones(3,3)  nHarmo=1  Measurements=None
  _CN_88916034_380000_CN_242756113_380000 : powerlib/Elements/Distributed Parameters Line  Phases=3  Frequency=50  Resistance=[0.01273 0.3864]  Inductance="[0.9337e-3  4.1264e-3]"  Capacitance=[12.74e-9 7.751e-9]  Length=131.6838  x1=[8.73114913702011e-11 380000 380000;314.159265358979 314.159265358979 314.159265358979;-0.177670123217348 0.415246442777429 -1.15554988401747]  x2=[1.26090477118469e-09 381852.398472139 381852.398472139;314.159265358979 314.159265358979 314.159265358979;-1.41941675517191 0.415007521738739 -1.15578880505616]  x3=[1.07663708898761e-11 1405.24743813465 1405.24743813466;314.159265358979 314.159265358979 314.159265358979;-2.70558821102223 0.316110507002444 -1.25468581979246]  x4=[8.62234243168895e-12 1405.96374414071 1405.9637441407;314.159265358979 314.159265358979 314.159265358979;0.245769282942371 0.405640215255436 -1.16515611153945]  x5=0.000565541566995742  V1=ones(3,3)  V2=ones(3,3)  I1=ones(3,3)  I2=ones(3,3)  nHarmo=1  Measurements=None
  _CN_88916034_380000_CN_25306752_380000 : powerlib/Elements/Distributed Parameters Line  Phases=3  Frequency=50  Resistance=[0.01273 0.3864]  Inductance="[0.9337e-3  4.1264e-3]"  Capacitance=[12.74e-9 7.751e-9]  Length=146.0141  x1=[8.73114913702011e-11 380000 380000;314.159265358979 314.159265358979 314.159265358979;-0.177670123217348 0.415246442777429 -1.15554988401747]  x2=[1.26090477118469e-09 381852.398472139 381852.398472139;314.159265358979 314.159265358979 314.159265358979;-1.41941675517191 0.415007521738739 -1.15578880505616]  x3=[1.07663708898761e-11 1405.24743813465 1405.24743813466;314.159265358979 314.159265358979 314.159265358979;-2.70558821102223 0.316110507002444 -1.25468581979246]  x4=[8.62234243168895e-12 1405.96374414071 1405.9637441407;314.159265358979 314.159265358979 314.159265358979;0.245769282942371 0.405640215255436 -1.16515611153945]  x5=0.000565541566995742  V1=ones(3,3)  V2=ones(3,3)  I1=ones(3,3)  I2=ones(3,3)  nHarmo=1  Measurements=None
  _CN_88916034_380000_CN_31367940_380000 : powerlib/Elements/Distributed Parameters Line  Phases=3  Frequency=50  Resistance=[0.01273 0.3864]  Inductance="[0.9337e-3  4.1264e-3]"  Capacitance=[12.74e-9 7.751e-9]  Length=44.3378  x1=[8.73114913702011e-11 380000 380000;314.159265358979 314.159265358979 314.159265358979;-0.177670123217348 0.415246442777429 -1.15554988401747]  x2=[1.26090477118469e-09 381852.398472139 381852.398472139;314.159265358979 314.159265358979 314.159265358979;-1.41941675517191 0.415007521738739 -1.15578880505616]  x3=[1.07663708898761e-11 1405.24743813465 1405.24743813466;314.159265358979 314.159265358979 314.159265358979;-2.70558821102223 0.316110507002444 -1.25468581979246]  x4=[8.62234243168895e-12 1405.96374414071 1405.9637441407;314.159265358979 314.159265358979 314.159265358979;0.245769282942371 0.405640215255436 -1.16515611153945]  x5=0.000565541566995742  V1=ones(3,3)  V2=ones(3,3)  I1=ones(3,3)  I2=ones(3,3)  nHarmo=1  Measurements=None
  _CN_88916034_380000_CN_35954395_380000 : powerlib/Elements/Distributed Parameters Line  Phases=3  Frequency=50  Resistance=[0.01273 0.3864]  Inductance="[0.9337e-3  4.1264e-3]"  Capacitance=[12.74e-9 7.751e-9]  Length=131.9598  x1=[8.73114913702011e-11 380000 380000;314.159265358979 314.159265358979 314.159265358979;-0.177670123217348 0.415246442777429 -1.15554988401747]  x2=[1.26090477118469e-09 381852.398472139 381852.398472139;314.159265358979 314.159265358979 314.159265358979;-1.41941675517191 0.415007521738739 -1.15578880505616]  x3=[1.07663708898761e-11 1405.24743813465 1405.24743813466;314.159265358979 314.159265358979 314.159265358979;-2.70558821102223 0.316110507002444 -1.25468581979246]  x4=[8.62234243168895e-12 1405.96374414071 1405.9637441407;314.159265358979 314.159265358979 314.159265358979;0.245769282942371 0.405640215255436 -1.16515611153945]  x5=0.000565541566995742  V1=ones(3,3)  V2=ones(3,3)  I1=ones(3,3)  I2=ones(3,3)  nHarmo=1  Measurements=None
  _CN_88916034_380000_CN_42049947_380000 : powerlib/Elements/Distributed Parameters Line  Phases=3  Frequency=50  Resistance=[0.01273 0.3864]  Inductance="[0.9337e-3  4.1264e-3]"  Capacitance=[12.74e-9 7.751e-9]  Length=125.6683  x1=[8.73114913702011e-11 380000 380000;314.159265358979 314.159265358979 314.159265358979;-0.177670123217348 0.415246442777429 -1.15554988401747]  x2=[1.26090477118469e-09 381852.398472139 381852.398472139;314.159265358979 314.159265358979 314.159265358979;-1.41941675517191 0.415007521738739 -1.15578880505616]  x3=[1.07663708898761e-11 1405.24743813465 1405.24743813466;314.159265358979 314.159265358979 314.159265358979;-2.70558821102223 0.316110507002444 -1.25468581979246]  x4=[8.62234243168895e-12 1405.96374414071 1405.9637441407;314.159265358979 314.159265358979 314.159265358979;0.245769282942371 0.405640215255436 -1.16515611153945]  x5=0.000565541566995742  V1=ones(3,3)  V2=ones(3,3)  I1=ones(3,3)  I2=ones(3,3)  nHarmo=1  Measurements=None
  _CN_88916034_380000_CN_42736239_380000 : powerlib/Elements/Distributed Parameters Line  Phases=3  Frequency=50  Resistance=[0.01273 0.3864]  Inductance="[0.9337e-3  4.1264e-3]"  Capacitance=[12.74e-9 7.751e-9]  Length=184.4985  x1=[8.73114913702011e-11 380000 380000;314.159265358979 314.159265358979 314.159265358979;-0.177670123217348 0.415246442777429 -1.15554988401747]  x2=[1.26090477118469e-09 381852.398472139 381852.398472139;314.159265358979 314.159265358979 314.159265358979;-1.41941675517191 0.415007521738739 -1.15578880505616]  x3=[1.07663708898761e-11 1405.24743813465 1405.24743813466;314.159265358979 314.159265358979 314.159265358979;-2.70558821102223 0.316110507002444 -1.25468581979246]  x4=[8.62234243168895e-12 1405.96374414071 1405.9637441407;314.159265358979 314.159265358979 314.159265358979;0.245769282942371 0.405640215255436 -1.16515611153945]  x5=0.000565541566995742  V1=ones(3,3)  V2=ones(3,3)  I1=ones(3,3)  I2=ones(3,3)  nHarmo=1  Measurements=None
  _CN_88916034_380000_CN_88901626_380000 : powerlib/Elements/Distributed Parameters Line  Phases=3  Frequency=50  Resistance=[0.01273 0.3864]  Inductance="[0.9337e-3  4.1264e-3]"  Capacitance=[12.74e-9 7.751e-9]  Length=34.7883  x1=[8.73114913702011e-11 380000 380000;314.159265358979 314.159265358979 314.159265358979;-0.177670123217348 0.415246442777429 -1.15554988401747]  x2=[1.26090477118469e-09 381852.398472139 381852.398472139;314.159265358979 314.159265358979 314.159265358979;-1.41941675517191 0.415007521738739 -1.15578880505616]  x3=[1.07663708898761e-11 1405.24743813465 1405.24743813466;314.159265358979 314.159265358979 314.159265358979;-2.70558821102223 0.316110507002444 -1.25468581979246]  x4=[8.62234243168895e-12 1405.96374414071 1405.9637441407;314.159265358979 314.159265358979 314.159265358979;0.245769282942371 0.405640215255436 -1.16515611153945]  x5=0.000565541566995742  V1=ones(3,3)  V2=ones(3,3)  I1=ones(3,3)  I2=ones(3,3)  nHarmo=1  Measurements=None
  _CN_88945213_380000_CN31023006 : powerlib/Elements/Distributed Parameters Line  Phases=3  Frequency=50  Resistance=[0.01273 0.3864]  Inductance="[0.9337e-3  4.1264e-3]"  Capacitance=[12.74e-9 7.751e-9]  Length=1.4124  x1=[8.73114913702011e-11 380000 380000;314.159265358979 314.159265358979 314.159265358979;-0.177670123217348 0.415246442777429 -1.15554988401747]  x2=[1.26090477118469e-09 381852.398472139 381852.398472139;314.159265358979 314.159265358979 314.159265358979;-1.41941675517191 0.415007521738739 -1.15578880505616]  x3=[1.07663708898761e-11 1405.24743813465 1405.24743813466;314.159265358979 314.159265358979 314.159265358979;-2.70558821102223 0.316110507002444 -1.25468581979246]  x4=[8.62234243168895e-12 1405.96374414071 1405.9637441407;314.159265358979 314.159265358979 314.159265358979;0.245769282942371 0.405640215255436 -1.16515611153945]  x5=0.000565541566995742  V1=ones(3,3)  V2=ones(3,3)  I1=ones(3,3)  I2=ones(3,3)  nHarmo=1  Measurements=None
  _CN_88945213_380000_CN_31019939_380000 : powerlib/Elements/Distributed Parameters Line  Phases=3  Frequency=50  Resistance=[0.01273 0.3864]  Inductance="[0.9337e-3  4.1264e-3]"  Capacitance=[12.74e-9 7.751e-9]  Length=3.3072  x1=[8.73114913702011e-11 380000 380000;314.159265358979 314.159265358979 314.159265358979;-0.177670123217348 0.415246442777429 -1.15554988401747]  x2=[1.26090477118469e-09 381852.398472139 381852.398472139;314.159265358979 314.159265358979 314.159265358979;-1.41941675517191 0.415007521738739 -1.15578880505616]  x3=[1.07663708898761e-11 1405.24743813465 1405.24743813466;314.159265358979 314.159265358979 314.159265358979;-2.70558821102223 0.316110507002444 -1.25468581979246]  x4=[8.62234243168895e-12 1405.96374414071 1405.9637441407;314.159265358979 314.159265358979 314.159265358979;0.245769282942371 0.405640215255436 -1.16515611153945]  x5=0.000565541566995742  V1=ones(3,3)  V2=ones(3,3)  I1=ones(3,3)  I2=ones(3,3)  nHarmo=1  Measurements=None
  _CN_89176939_220000_CN_151967290_220000 : powerlib/Elements/Distributed Parameters Line  Phases=3  Frequency=50  Resistance=[0.01273 0.3864]  Inductance="[0.9337e-3  4.1264e-3]"  Capacitance=[12.74e-9 7.751e-9]  Length=31.7398  x1=[8.73114913702011e-11 380000 380000;314.159265358979 314.159265358979 314.159265358979;-0.177670123217348 0.415246442777429 -1.15554988401747]  x2=[1.26090477118469e-09 381852.398472139 381852.398472139;314.159265358979 314.159265358979 314.159265358979;-1.41941675517191 0.415007521738739 -1.15578880505616]  x3=[1.07663708898761e-11 1405.24743813465 1405.24743813466;314.159265358979 314.159265358979 314.159265358979;-2.70558821102223 0.316110507002444 -1.25468581979246]  x4=[8.62234243168895e-12 1405.96374414071 1405.9637441407;314.159265358979 314.159265358979 314.159265358979;0.245769282942371 0.405640215255436 -1.16515611153945]  x5=0.000565541566995742  V1=ones(3,3)  V2=ones(3,3)  I1=ones(3,3)  I2=ones(3,3)  nHarmo=1  Measurements=None
  _CN_89176939_220000_CN_89176956_220000 : powerlib/Elements/Distributed Parameters Line  Phases=3  Frequency=50  Resistance=[0.01273 0.3864]  Inductance="[0.9337e-3  4.1264e-3]"  Capacitance=[12.74e-9 7.751e-9]  Length=3.9596  x1=[8.73114913702011e-11 380000 380000;314.159265358979 314.159265358979 314.159265358979;-0.177670123217348 0.415246442777429 -1.15554988401747]  x2=[1.26090477118469e-09 381852.398472139 381852.398472139;314.159265358979 314.159265358979 314.159265358979;-1.41941675517191 0.415007521738739 -1.15578880505616]  x3=[1.07663708898761e-11 1405.24743813465 1405.24743813466;314.159265358979 314.159265358979 314.159265358979;-2.70558821102223 0.316110507002444 -1.25468581979246]  x4=[8.62234243168895e-12 1405.96374414071 1405.9637441407;314.159265358979 314.159265358979 314.159265358979;0.245769282942371 0.405640215255436 -1.16515611153945]  x5=0.000565541566995742  V1=ones(3,3)  V2=ones(3,3)  I1=ones(3,3)  I2=ones(3,3)  nHarmo=1  Measurements=None
  _CN_89215122_220000_CN_145680894_220000 : powerlib/Elements/Distributed Parameters Line  Phases=3  Frequency=50  Resistance=[0.01273 0.3864]  Inductance="[0.9337e-3  4.1264e-3]"  Capacitance=[12.74e-9 7.751e-9]  Length=91.7856  x1=[8.73114913702011e-11 380000 380000;314.159265358979 314.159265358979 314.159265358979;-0.177670123217348 0.415246442777429 -1.15554988401747]  x2=[1.26090477118469e-09 381852.398472139 381852.398472139;314.159265358979 314.159265358979 314.159265358979;-1.41941675517191 0.415007521738739 -1.15578880505616]  x3=[1.07663708898761e-11 1405.24743813465 1405.24743813466;314.159265358979 314.159265358979 314.159265358979;-2.70558821102223 0.316110507002444 -1.25468581979246]  x4=[8.62234243168895e-12 1405.96374414071 1405.9637441407;314.159265358979 314.159265358979 314.159265358979;0.245769282942371 0.405640215255436 -1.16515611153945]  x5=0.000565541566995742  V1=ones(3,3)  V2=ones(3,3)  I1=ones(3,3)  I2=ones(3,3)  nHarmo=1  Measurements=None
  _CN_89215122_220000_CN_54359256_220000 : powerlib/Elements/Distributed Parameters Line  Phases=3  Frequency=50  Resistance=[0.01273 0.3864]  Inductance="[0.9337e-3  4.1264e-3]"  Capacitance=[12.74e-9 7.751e-9]  Length=34.8189  x1=[8.73114913702011e-11 380000 380000;314.159265358979 314.159265358979 314.159265358979;-0.177670123217348 0.415246442777429 -1.15554988401747]  x2=[1.26090477118469e-09 381852.398472139 381852.398472139;314.159265358979 314.159265358979 314.159265358979;-1.41941675517191 0.415007521738739 -1.15578880505616]  x3=[1.07663708898761e-11 1405.24743813465 1405.24743813466;314.159265358979 314.159265358979 314.159265358979;-2.70558821102223 0.316110507002444 -1.25468581979246]  x4=[8.62234243168895e-12 1405.96374414071 1405.9637441407;314.159265358979 314.159265358979 314.159265358979;0.245769282942371 0.405640215255436 -1.16515611153945]  x5=0.000565541566995742  V1=ones(3,3)  V2=ones(3,3)  I1=ones(3,3)  I2=ones(3,3)  nHarmo=1  Measurements=None
  _CN_89215122_220000_CN_82310607_220000 : powerlib/Elements/Distributed Parameters Line  Phases=3  Frequency=50  Resistance=[0.01273 0.3864]  Inductance="[0.9337e-3  4.1264e-3]"  Capacitance=[12.74e-9 7.751e-9]  Length=15.8945  x1=[8.73114913702011e-11 380000 380000;314.159265358979 314.159265358979 314.159265358979;-0.177670123217348 0.415246442777429 -1.15554988401747]  x2=[1.26090477118469e-09 381852.398472139 381852.398472139;314.159265358979 314.159265358979 314.159265358979;-1.41941675517191 0.415007521738739 -1.15578880505616]  x3=[1.07663708898761e-11 1405.24743813465 1405.24743813466;314.159265358979 314.159265358979 314.159265358979;-2.70558821102223 0.316110507002444 -1.25468581979246]  x4=[8.62234243168895e-12 1405.96374414071 1405.9637441407;314.159265358979 314.159265358979 314.159265358979;0.245769282942371 0.405640215255436 -1.16515611153945]  x5=0.000565541566995742  V1=ones(3,3)  V2=ones(3,3)  I1=ones(3,3)  I2=ones(3,3)  nHarmo=1  Measurements=None
  _CN_89352550_220000_CN28051874 : powerlib/Elements/Distributed Parameters Line  Phases=3  Frequency=50  Resistance=[0.01273 0.3864]  Inductance="[0.9337e-3  4.1264e-3]"  Capacitance=[12.74e-9 7.751e-9]  Length=0.064891  x1=[8.73114913702011e-11 380000 380000;314.159265358979 314.159265358979 314.159265358979;-0.177670123217348 0.415246442777429 -1.15554988401747]  x2=[1.26090477118469e-09 381852.398472139 381852.398472139;314.159265358979 314.159265358979 314.159265358979;-1.41941675517191 0.415007521738739 -1.15578880505616]  x3=[1.07663708898761e-11 1405.24743813465 1405.24743813466;314.159265358979 314.159265358979 314.159265358979;-2.70558821102223 0.316110507002444 -1.25468581979246]  x4=[8.62234243168895e-12 1405.96374414071 1405.9637441407;314.159265358979 314.159265358979 314.159265358979;0.245769282942371 0.405640215255436 -1.16515611153945]  x5=0.000565541566995742  V1=ones(3,3)  V2=ones(3,3)  I1=ones(3,3)  I2=ones(3,3)  nHarmo=1  Measurements=None
  _CN_89352550_380000_CN28051874 : powerlib/Elements/Distributed Parameters Line  Phases=3  Frequency=50  Resistance=[0.01273 0.3864]  Inductance="[0.9337e-3  4.1264e-3]"  Capacitance=[12.74e-9 7.751e-9]  Length=0.38654  x1=[8.73114913702011e-11 380000 380000;314.159265358979 314.159265358979 314.159265358979;-0.177670123217348 0.415246442777429 -1.15554988401747]  x2=[1.26090477118469e-09 381852.398472139 381852.398472139;314.159265358979 314.159265358979 314.159265358979;-1.41941675517191 0.415007521738739 -1.15578880505616]  x3=[1.07663708898761e-11 1405.24743813465 1405.24743813466;314.159265358979 314.159265358979 314.159265358979;-2.70558821102223 0.316110507002444 -1.25468581979246]  x4=[8.62234243168895e-12 1405.96374414071 1405.9637441407;314.159265358979 314.159265358979 314.159265358979;0.245769282942371 0.405640215255436 -1.16515611153945]  x5=0.000565541566995742  V1=ones(3,3)  V2=ones(3,3)  I1=ones(3,3)  I2=ones(3,3)  nHarmo=1  Measurements=None
  _CN_90109302_220000_CN_82310607_220000 : powerlib/Elements/Distributed Parameters Line  Phases=3  Frequency=50  Resistance=[0.01273 0.3864]  Inductance="[0.9337e-3  4.1264e-3]"  Capacitance=[12.74e-9 7.751e-9]  Length=0.74181  x1=[8.73114913702011e-11 380000 380000;314.159265358979 314.159265358979 314.159265358979;-0.177670123217348 0.415246442777429 -1.15554988401747]  x2=[1.26090477118469e-09 381852.398472139 381852.398472139;314.159265358979 314.159265358979 314.159265358979;-1.41941675517191 0.415007521738739 -1.15578880505616]  x3=[1.07663708898761e-11 1405.24743813465 1405.24743813466;314.159265358979 314.159265358979 314.159265358979;-2.70558821102223 0.316110507002444 -1.25468581979246]  x4=[8.62234243168895e-12 1405.96374414071 1405.9637441407;314.159265358979 314.159265358979 314.159265358979;0.245769282942371 0.405640215255436 -1.16515611153945]  x5=0.000565541566995742  V1=ones(3,3)  V2=ones(3,3)  I1=ones(3,3)  I2=ones(3,3)  nHarmo=1  Measurements=None
  _CN_91080806_220000_CN167578660 : powerlib/Elements/Distributed Parameters Line  Phases=3  Frequency=50  Resistance=[0.01273 0.3864]  Inductance="[0.9337e-3  4.1264e-3]"  Capacitance=[12.74e-9 7.751e-9]  Length=0.22482  x1=[8.73114913702011e-11 380000 380000;314.159265358979 314.159265358979 314.159265358979;-0.177670123217348 0.415246442777429 -1.15554988401747]  x2=[1.26090477118469e-09 381852.398472139 381852.398472139;314.159265358979 314.159265358979 314.159265358979;-1.41941675517191 0.415007521738739 -1.15578880505616]  x3=[1.07663708898761e-11 1405.24743813465 1405.24743813466;314.159265358979 314.159265358979 314.159265358979;-2.70558821102223 0.316110507002444 -1.25468581979246]  x4=[8.62234243168895e-12 1405.96374414071 1405.9637441407;314.159265358979 314.159265358979 314.159265358979;0.245769282942371 0.405640215255436 -1.16515611153945]  x5=0.000565541566995742  V1=ones(3,3)  V2=ones(3,3)  I1=ones(3,3)  I2=ones(3,3)  nHarmo=1  Measurements=None
  _CN_91086220_220000_CN167578660 : powerlib/Elements/Distributed Parameters Line  Phases=3  Frequency=50  Resistance=[0.01273 0.3864]  Inductance="[0.9337e-3  4.1264e-3]"  Capacitance=[12.74e-9 7.751e-9]  Length=58.0713  x1=[8.73114913702011e-11 380000 380000;314.159265358979 314.159265358979 314.159265358979;-0.177670123217348 0.415246442777429 -1.15554988401747]  x2=[1.26090477118469e-09 381852.398472139 381852.398472139;314.159265358979 314.159265358979 314.159265358979;-1.41941675517191 0.415007521738739 -1.15578880505616]  x3=[1.07663708898761e-11 1405.24743813465 1405.24743813466;314.159265358979 314.159265358979 314.159265358979;-2.70558821102223 0.316110507002444 -1.25468581979246]  x4=[8.62234243168895e-12 1405.96374414071 1405.9637441407;314.159265358979 314.159265358979 314.159265358979;0.245769282942371 0.405640215255436 -1.16515611153945]  x5=0.000565541566995742  V1=ones(3,3)  V2=ones(3,3)  I1=ones(3,3)  I2=ones(3,3)  nHarmo=1  Measurements=None
  _CN_91086220_220000_CN_24976300_220000 : powerlib/Elements/Distributed Parameters Line  Phases=3  Frequency=50  Resistance=[0.01273 0.3864]  Inductance="[0.9337e-3  4.1264e-3]"  Capacitance=[12.74e-9 7.751e-9]  Length=83.4577  x1=[8.73114913702011e-11 380000 380000;314.159265358979 314.159265358979 314.159265358979;-0.177670123217348 0.415246442777429 -1.15554988401747]  x2=[1.26090477118469e-09 381852.398472139 381852.398472139;314.159265358979 314.159265358979 314.159265358979;-1.41941675517191 0.415007521738739 -1.15578880505616]  x3=[1.07663708898761e-11 1405.24743813465 1405.24743813466;314.159265358979 314.159265358979 314.159265358979;-2.70558821102223 0.316110507002444 -1.25468581979246]  x4=[8.62234243168895e-12 1405.96374414071 1405.9637441407;314.159265358979 314.159265358979 314.159265358979;0.245769282942371 0.405640215255436 -1.16515611153945]  x5=0.000565541566995742  V1=ones(3,3)  V2=ones(3,3)  I1=ones(3,3)  I2=ones(3,3)  nHarmo=1  Measurements=None
  _CN_91086220_220000_CN_77694901_220000 : powerlib/Elements/Distributed Parameters Line  Phases=3  Frequency=50  Resistance=[0.01273 0.3864]  Inductance="[0.9337e-3  4.1264e-3]"  Capacitance=[12.74e-9 7.751e-9]  Length=111.814  x1=[8.73114913702011e-11 380000 380000;314.159265358979 314.159265358979 314.159265358979;-0.177670123217348 0.415246442777429 -1.15554988401747]  x2=[1.26090477118469e-09 381852.398472139 381852.398472139;314.159265358979 314.159265358979 314.159265358979;-1.41941675517191 0.415007521738739 -1.15578880505616]  x3=[1.07663708898761e-11 1405.24743813465 1405.24743813466;314.159265358979 314.159265358979 314.159265358979;-2.70558821102223 0.316110507002444 -1.25468581979246]  x4=[8.62234243168895e-12 1405.96374414071 1405.9637441407;314.159265358979 314.159265358979 314.159265358979;0.245769282942371 0.405640215255436 -1.16515611153945]  x5=0.000565541566995742  V1=ones(3,3)  V2=ones(3,3)  I1=ones(3,3)  I2=ones(3,3)  nHarmo=1  Measurements=None
  powergui : powerlib/powergui  Priority=1  SimulationMode=Phasor  SolverType=Tustin/Backward Euler (TBE)  SampleTime=50e-6  frequency=50  SPID=off  DisableSnubberDevices=off  DisableRonSwitches=off  DisableVfSwitches=off  SwTol=0  DisplayEquations=off  Interpol=off  ExternalGateDelay=off  methode=off  Ts=10  FunctionMessages=off  echomessages=off  HookPort=off  EnableUseOfTLC=off  x0status=blocks  frequencyindice=50  Pbase=3000e6  ErrMax=0.0001  Iterations=50  UnitsV=V  UnitsW=W  buscounter=0  RestoreLinks=warning  ResistiveCurrentMeasurement=off  Frange=[0:2:500]  Ylog=off  Xlog=on  ShowGrid=off  save=off  variable=ZData  structure=0  ZoomFFT=off  StartTime=0.0  cycles=1  DisplayStyle=1  fundamental=60  FreqAxis=off  MaxFrequency=1000  frequencyindicesteady=1  RmsSteady=1  display=off
  Öldruckkabel_CN_202865176_220000_CN129989100 : powerlib/Elements/Distributed Parameters Line  Phases=3  Frequency=50  Resistance=[0.01273 0.3864]  Inductance="[0.9337e-3  4.1264e-3]"  Capacitance=[12.74e-9 7.751e-9]  Length=0.97449  x1=[8.73114913702011e-11 380000 380000;314.159265358979 314.159265358979 314.159265358979;-0.177670123217348 0.415246442777429 -1.15554988401747]  x2=[1.26090477118469e-09 381852.398472139 381852.398472139;314.159265358979 314.159265358979 314.159265358979;-1.41941675517191 0.415007521738739 -1.15578880505616]  x3=[1.07663708898761e-11 1405.24743813465 1405.24743813466;314.159265358979 314.159265358979 314.159265358979;-2.70558821102223 0.316110507002444 -1.25468581979246]  x4=[8.62234243168895e-12 1405.96374414071 1405.9637441407;314.159265358979 314.159265358979 314.159265358979;0.245769282942371 0.405640215255436 -1.16515611153945]  x5=0.000565541566995742  V1=ones(3,3)  V2=ones(3,3)  I1=ones(3,3)  I2=ones(3,3)  nHarmo=1  Measurements=None
  connections:
  Hattorf_2_CN_24262656_380000_CN_24258096_380000/LConn1 -- T_24262656_380000;220000_Wahle/LConn1 -- Leitung_3026_CN_24262656_380000_CN_23899043_380000/LConn1 -- Leitung_3026_CN_24262656_380000_CN23773034/LConn1 -- Leitung_3026_CN_24262656_380000_CN_24413992_380000/LConn1 -- Leitung_3026_CN_24262656_380000_CN_24272339_380000/LConn1 -- Stadorf_1_CN_24262656_380000_CN_28343121_380000/LConn1
  Hattorf_2_CN_24262656_380000_CN_24258096_380000/LConn2 -- T_24262656_380000;220000_Wahle/LConn2 -- Leitung_3026_CN_24262656_380000_CN_23899043_380000/LConn2 -- Leitung_3026_CN_24262656_380000_CN23773034/LConn2 -- Leitung_3026_CN_24262656_380000_CN_24413992_380000/LConn2 -- Leitung_3026_CN_24262656_380000_CN_24272339_380000/LConn2 -- Stadorf_1_CN_24262656_380000_CN_28343121_380000/LConn2
  Hattorf_2_CN_24262656_380000_CN_24258096_380000/LConn3 -- T_24262656_380000;220000_Wahle/LConn3 -- Leitung_3026_CN_24262656_380000_CN_23899043_380000/LConn3 -- Leitung_3026_CN_24262656_380000_CN23773034/LConn3 -- Leitung_3026_CN_24262656_380000_CN_24413992_380000/LConn3 -- Leitung_3026_CN_24262656_380000_CN_24272339_380000/LConn3 -- Stadorf_1_CN_24262656_380000_CN_28343121_380000/LConn3
  Hattorf_2_CN_24262656_380000_CN_24258096_380000/RConn1 -- T_24258096_380000_Umspannwerk_Hattorf/LConn1 -- Helmstedt_380_kV_CN_26474759_380000_CN_24258096_380000/LConn1
  Hattorf_2_CN_24262656_380000_CN_24258096_380000/RConn2 -- T_24258096_380000_Umspannwerk_Hattorf/LConn2 -- Helmstedt_380_kV_CN_26474759_380000_CN_24258096_380000/LConn2
  Hattorf_2_CN_24262656_380000_CN_24258096_380000/RConn3 -- T_24258096_380000_Umspannwerk_Hattorf/LConn3 -- Helmstedt_380_kV_CN_26474759_380000_CN_24258096_380000/LConn3
  Gleidingen_2_CN_24262656_220000_CN_30017786_220000/LConn1 -- T_24262656_380000;220000_Wahle/RConn1 -- Braunschweig_Nord_1_CN_24262656_220000_CN_24272541_220000/LConn1 -- L_24262656/LConn1 -- Gleidingen_2_CN_24262656_220000_CN_28227099_220000/LConn1 -- Gleidingen_2_CN_24262656_220000_CN23681460/LConn1
  Gleidingen_2_CN_24262656_220000_CN_30017786_220000/LConn2 -- T_24262656_380000;220000_Wahle/RConn2 -- Braunschweig_Nord_1_CN_24262656_220000_CN_24272541_220000/LConn2 -- L_24262656/LConn2 -- Gleidingen_2_CN_24262656_220000_CN_28227099_220000/LConn2 -- Gleidingen_2_CN_24262656_220000_CN23681460/LConn2
  Gleidingen_2_CN_24262656_220000_CN_30017786_220000/LConn3 -- T_24262656_380000;220000_Wahle/RConn3 -- Braunschweig_Nord_1_CN_24262656_220000_CN_24272541_220000/LConn3 -- L_24262656/LConn3 -- Gleidingen_2_CN_24262656_220000_CN_28227099_220000/LConn3 -- Gleidingen_2_CN_24262656_220000_CN23681460/LConn3
  T_30017786_220000_Gleidingen_220_kV/LConn1 -- Gleidingen_2_CN_24262656_220000_CN_30017786_220000/RConn1
  T_30017786_220000_Gleidingen_220_kV/LConn2 -- Gleidingen_2_CN_24262656_220000_CN_30017786_220000/RConn2
  T_30017786_220000_Gleidingen_220_kV/LConn3 -- Gleidingen_2_CN_24262656_220000_CN_30017786_220000/RConn3
  Gleidingen_2_CN_24262656_220000_CN_28227099_220000/RConn1 -- _CN_151507370_220000_CN_28227099_220000/LConn1 -- _CN_28227099_220000_CN_97857512_220000/LConn1 -- T_28227099_220000;110000_Salzgitter_Hallendorf/LConn1
  Gleidingen_2_CN_24262656_220000_CN_28227099_220000/RConn2 -- T_28227099_220000;110000_Salzgitter_Hallendorf/LConn2 -- _CN_151507370_220000_CN_28227099_220000/LConn2 -- _CN_28227099_220000_CN_97857512_220000/LConn2
  Gleidingen_2_CN_24262656_220000_CN_28227099_220000/RConn3 -- T_28227099_220000;110000_Salzgitter_Hallendorf/LConn3 -- _CN_151507370_220000_CN_28227099_220000/LConn3 -- _CN_28227099_220000_CN_97857512_220000/LConn3
  Gleidingen_2_CN_24262656_220000_CN23681460/RConn1 -- G_23681460_Gemeinschaftskraftwerk_Mehrum/RConn1 -- Leitung_2026_CN_33042984_220000_CN23681460/LConn1 -- Salzgitter_Hallendorf_CN_274621059_220000_CN23681460/LConn1 -- _CN_23816140_220000_CN23681460/LConn1
  Gleidingen_2_CN_24262656_220000_CN23681460/RConn2 -- G_23681460_Gemeinschaftskraftwerk_Mehrum/RConn2 -- Leitung_2026_CN_33042984_220000_CN23681460/LConn2 -- Salzgitter_Hallendorf_CN_274621059_220000_CN23681460/LConn2 -- _CN_23816140_220000_CN23681460/LConn2
  Gleidingen_2_CN_24262656_220000_CN23681460/RConn3 -- G_23681460_Gemeinschaftskraftwerk_Mehrum/RConn3 -- Leitung_2026_CN_33042984_220000_CN23681460/LConn3 -- Salzgitter_Hallendorf_CN_274621059_220000_CN23681460/LConn3 -- _CN_23816140_220000_CN23681460/LConn3
  T_23899043_380000;110000_Algermissen/LConn1 -- Leitung_3026_CN_24262656_380000_CN_23899043_380000/RConn1
  T_23899043_380000;110000_Algermissen/LConn2 -- Leitung_3026_CN_24262656_380000_CN_23899043_380000/RConn2
  T_23899043_380000;110000_Algermissen/LConn3 -- Leitung_3026_CN_24262656_380000_CN_23899043_380000/RConn3
  Leitung_3026_CN_24262656_380000_CN23773034/RConn1 -- G_23773034_Kernkraftwerk_Grohnde/RConn1 -- Leitung_3013_CN_24413992_380000_CN23773034/LConn1
  Leitung_3026_CN_24262656_380000_CN23773034/RConn2 -- G_23773034_Kernkraftwerk_Grohnde/RConn2 -- Leitung_3013_CN_24413992_380000_CN23773034/LConn2
  Leitung_3026_CN_24262656_380000_CN23773034/RConn3 -- G_23773034_Kernkraftwerk_Grohnde/RConn3 -- Leitung_3013_CN_24413992_380000_CN23773034/LConn3
  Leitung_3026_CN_24262656_380000_CN_24413992_380000/RConn1 -- T_24413992_380000;110000_UW_Grohnde_380_kV___110_kV/LConn1 -- _CN_42681484_380000_CN_24413992_380000/LConn1 -- Leitung_3011_CN_27739871_380000_CN_24413992_380000/LConn1 -- Leitung_3013_CN_24413992_380000_CN23773034/RConn1
  Leitung_3026_CN_24262656_380000_CN_24413992_380000/RConn2 -- T_24413992_380000;110000_UW_Grohnde_380_kV___110_kV/LConn2 -- _CN_42681484_380000_CN_24413992_380000/LConn2 -- Leitung_3011_CN_27739871_380000_CN_24413992_380000/LConn2 -- Leitung_3013_CN_24413992_380000_CN23773034/RConn2
  Leitung_3026_CN_24262656_380000_CN_24413992_380000/RConn3 -- T_24413992_380000;110000_UW_Grohnde_380_kV___110_kV/LConn3 -- _CN_42681484_380000_CN_24413992_380000/LConn3 -- Leitung_3011_CN_27739871_380000_CN_24413992_380000/LConn3 -- Leitung_3013_CN_24413992_380000_CN23773034/RConn3
  T_24272339_380000;110000_Klein_Ilsede/LConn1 -- Leitung_3026_CN_24262656_380000_CN_24272339_380000/RConn1
  T_24272339_380000;110000_Klein_Ilsede/LConn2 -- Leitung_3026_CN_24262656_380000_CN_24272339_380000/RConn2
  T_24272339_380000;110000_Klein_Ilsede/LConn3 -- Leitung_3026_CN_24262656_380000_CN_24272339_380000/RConn3
  T_24272541_220000_Umspannwerk_Braunschweig_Nord/LConn1 -- Braunschweig_Nord_1_CN_24262656_220000_CN_24272541_220000/RConn1
  T_24272541_220000_Umspannwerk_Braunschweig_Nord/LConn2 -- Braunschweig_Nord_1_CN_24262656_220000_CN_24272541_220000/RConn2
  T_24272541_220000_Umspannwerk_Braunschweig_Nord/LConn3 -- Braunschweig_Nord_1_CN_24262656_220000_CN_24272541_220000/RConn3
  Stadorf_1_CN_24262656_380000_CN_28343121_380000/RConn1 -- T_28343121_380000_Stadorf/LConn1 -- 3021_UW_Lüneburg___UW_Stadorf_CN_28343121_380000_CN_28327356_380000/LConn1
  Stadorf_1_CN_24262656_380000_CN_28343121_380000/RConn2 -- T_28343121_380000_Stadorf/LConn2 -- 3021_UW_Lüneburg___UW_Stadorf_CN_28343121_380000_CN_28327356_380000/LConn2
  Stadorf_1_CN_24262656_380000_CN_28343121_380000/RConn3 -- T_28343121_380000_Stadorf/LConn3 -- 3021_UW_Lüneburg___UW_Stadorf_CN_28343121_380000_CN_28327356_380000/LConn3
  _CN_41334805_220000_CN_25786404_220000/LConn1 -- T_41334805_220000_Drehstromschaltwerk_Neckarwestheim/LConn1 -- _CN_41334805_220000_CN_43688805_220000/LConn1 -- _CN_41334805_220000_CN_23414063_220000/LConn1 -- _CN_41334805_220000_CN_143903369_220000/LConn1 -- _CN_41334805_220000_CN_152973139_220000/LConn1 -- _CN_41334805_220000_CN_207248812_220000/LConn1 -- _CN_41334805_220000_CN_25557397_220000/LConn1 -- Anlage_373_CN_41334805_220000_CN23547196/LConn1
  _CN_41334805_220000_CN_25786404_220000/LConn2 -- T_41334805_220000_Drehstromschaltwerk_Neckarwestheim/LConn2 -- _CN_41334805_220000_CN_43688805_220000/LConn2 -- _CN_41334805_220000_CN_23414063_220000/LConn2 -- _CN_41334805_220000_CN_143903369_220000/LConn2 -- _CN_41334805_220000_CN_152973139_220000/LConn2 -- _CN_41334805_220000_CN_207248812_220000/LConn2 -- _CN_41334805_220000_CN_25557397_220000/LConn2 -- Anlage_373_CN_41334805_220000_CN23547196/LConn2
  _CN_41334805_220000_CN_25786404_220000/LConn3 -- T_41334805_220000_Drehstromschaltwerk_Neckarwestheim/LConn3 -- _CN_41334805_220000_CN_43688805_220000/LConn3 -- _CN_41334805_220000_CN_23414063_220000/LConn3 -- _CN_41334805_220000_CN_143903369_220000/LConn3 -- _CN_41334805_220000_CN_152973139_220000/LConn3 -- _CN_41334805_220000_CN_207248812_220000/LConn3 -- _CN_41334805_220000_CN_25557397_220000/LConn3 -- Anlage_373_CN_41334805_220000_CN23547196/LConn3
  _CN_41334805_220000_CN_25786404_220000/RConn1 -- T_25786404_220000;110000_Umspannwerk_Hoheneck_EnBW/LConn1 -- Anlage_322_CN_25786404_220000_CN_97825259_220000/LConn1 -- Anlage_322_CN_25786404_220000_CN_32205824_220000/LConn1 -- Anlage_322_CN_25786404_220000_CN_26260052_220000/LConn1 -- _CN_25786404_220000_CN_25802269_220000/LConn1 -- Anlage_4508_CN_25786404_220000_CN_25306752_220000/LConn1
  _CN_41334805_220000_CN_25786404_220000/RConn2 -- T_25786404_220000;110000_Umspannwerk_Hoheneck_EnBW/LConn2 -- Anlage_322_CN_25786404_220000_CN_97825259_220000/LConn2 -- Anlage_322_CN_25786404_220000_CN_32205824_220000/LConn2 -- Anlage_322_CN_25786404_220000_CN_26260052_220000/LConn2 -- _CN_25786404_220000_CN_25802269_220000/LConn2 -- Anlage_4508_CN_25786404_220000_CN_25306752_220000/LConn2
  _CN_41334805_220000_CN_25786404_220000/RConn3 -- T_25786404_220000;110000_Umspannwerk_Hoheneck_EnBW/LConn3 -- Anlage_322_CN_25786404_220000_CN_97825259_220000/LConn3 -- Anlage_322_CN_25786404_220000_CN_32205824_220000/LConn3 -- Anlage_322_CN_25786404_220000_CN_26260052_220000/LConn3 -- _CN_25786404_220000_CN_25802269_220000/LConn3 -- Anlage_4508_CN_25786404_220000_CN_25306752_220000/LConn3
  _CN_41334805_220000_CN_43688805_220000/RConn1 -- T_43688805_380000;220000;110000_380kV_Umspannwerk_Pulverdingen/RConn1 -- L_43688805/LConn1
  _CN_41334805_220000_CN_43688805_220000/RConn2 -- T_43688805_380000;220000;110000_380kV_Umspannwerk_Pulverdingen/RConn2 -- L_43688805/LConn2
  _CN_41334805_220000_CN_43688805_220000/RConn3 -- T_43688805_380000;220000;110000_380kV_Umspannwerk_Pulverdingen/RConn3 -- L_43688805/LConn3
  T_23414063_220000;110000_Umspannwerk_Weilimdorf/LConn1 -- _CN_41334805_220000_CN_23414063_220000/RConn1
  T_23414063_220000;110000_Umspannwerk_Weilimdorf/LConn2 -- _CN_41334805_220000_CN_23414063_220000/RConn2
  T_23414063_220000;110000_Umspannwerk_Weilimdorf/LConn3 -- _CN_41334805_220000_CN_23414063_220000/RConn3
  _CN_41334805_220000_CN_143903369_220000/RConn1 -- T_143903369_380000;220000;110000_Umspannwerk_Hüffenhardt/RConn1 -- _CN_25557397_220000_CN_143903369_220000/LConn1 -- L_143903369/LConn1
  _CN_41334805_220000_CN_143903369_220000/RConn2 -- T_143903369_380000;220000;110000_Umspannwerk_Hüffenhardt/RConn2 -- _CN_25557397_220000_CN_143903369_220000/LConn2 -- L_143903369/LConn2
  _CN_41334805_220000_CN_143903369_220000/RConn3 -- T_143903369_380000;220000;110000_Umspannwerk_Hüffenhardt/RConn3 -- _CN_25557397_220000_CN_143903369_220000/LConn3 -- L_143903369/LConn3
  _CN_41334805_220000_CN_152973139_220000/RConn1 -- T_152973139_220000;110000_Station_Rheinau/LConn1 -- 220_kV_Rheinau_Ost|West_CN_147521567_220000_CN_152973139_220000/LConn1
  _CN_41334805_220000_CN_152973139_220000/RConn2 -- T_152973139_220000;110000_Station_Rheinau/LConn2 -- 220_kV_Rheinau_Ost|West_CN_147521567_220000_CN_152973139_220000/LConn2
  _CN_41334805_220000_CN_152973139_220000/RConn3 -- T_152973139_220000;110000_Station_Rheinau/LConn3 -- 220_kV_Rheinau_Ost|West_CN_147521567_220000_CN_152973139_220000/LConn3
  _CN_41334805_220000_CN_207248812_220000/RConn1 -- T_207248812_380000;220000_Umspannwerk_Neurott/RConn1 -- _CN_152261133_220000_CN_207248812_220000/LConn1 -- _CN_207248812_220000_CN_156676050_220000/LConn1 -- L_207248812/LConn1
  _CN_41334805_220000_CN_207248812_220000/RConn2 -- T_207248812_380000;220000_Umspannwerk_Neurott/RConn2 -- _CN_152261133_220000_CN_207248812_220000/LConn2 -- _CN_207248812_220000_CN_156676050_220000/LConn2 -- L_207248812/LConn2
  _CN_41334805_220000_CN_207248812_220000/RConn3 -- T_207248812_380000;220000_Umspannwerk_Neurott/RConn3 -- _CN_152261133_220000_CN_207248812_220000/LConn3 -- _CN_207248812_220000_CN_156676050_220000/LConn3 -- L_207248812/LConn3
  _CN_41334805_220000_CN_25557397_220000/RConn1 -- T_25557397_380000;220000;110000_380_kV_Umspannwerk_Großgartach/RConn1 -- _CN_25557397_220000_CN_42050342_220000/LConn1 -- _CN_25557397_220000_CN89183108/LConn1 -- L_25557397/LConn1 -- _CN_25557397_220000_CN146723308/LConn1 -- _CN_25557397_220000_CN_143903369_220000/RConn1
  _CN_41334805_220000_CN_25557397_220000/RConn2 -- T_25557397_380000;220000;110000_380_kV_Umspannwerk_Großgartach/RConn2 -- _CN_25557397_220000_CN_42050342_220000/LConn2 -- _CN_25557397_220000_CN89183108/LConn2 -- L_25557397/LConn2 -- _CN_25557397_220000_CN146723308/LConn2 -- _CN_25557397_220000_CN_143903369_220000/RConn2
  _CN_41334805_220000_CN_25557397_220000/RConn3 -- T_25557397_380000;220000;110000_380_kV_Umspannwerk_Großgartach/RConn3 -- _CN_25557397_220000_CN_42050342_220000/LConn3 -- _CN_25557397_220000_CN89183108/LConn3 -- L_25557397/LConn3 -- _CN_25557397_220000_CN146723308/LConn3 -- _CN_25557397_220000_CN_143903369_220000/RConn3
  Anlage_373_CN_41334805_220000_CN23547196/RConn1 -- G_23547196_Gemeinschaftskraftwerk_Neckarwestheim/RConn1 -- _CN_25557397_380000_CN23547196/LConn1 -- _CN_147878692_380000_CN23547196/LConn1 -- _CN_153328698_380000_CN23547196/LConn1
  Anlage_373_CN_41334805_220000_CN23547196/RConn2 -- G_23547196_Gemeinschaftskraftwerk_Neckarwestheim/RConn2 -- _CN_25557397_380000_CN23547196/LConn2 -- _CN_147878692_380000_CN23547196/LConn2 -- _CN_153328698_380000_CN23547196/LConn2
  Anlage_373_CN_41334805_220000_CN23547196/RConn3 -- G_23547196_Gemeinschaftskraftwerk_Neckarwestheim/RConn3 -- _CN_25557397_380000_CN23547196/LConn3 -- _CN_147878692_380000_CN23547196/LConn3 -- _CN_153328698_380000_CN23547196/LConn3
  Markersbach_Zwönitz_Röhrsdorf_CN_166604822_380000_CN_23117075_380000/LConn1 -- T_166604822_380000_Markersbach/LConn1 -- Markersbach_Zwönitz_Röhrsdorf_CN_166604822_380000_CN_36183042_380000/LConn1
  Markersbach_Zwönitz_Röhrsdorf_CN_166604822_380000_CN_23117075_380000/LConn2 -- T_166604822_380000_Markersbach/LConn2 -- Markersbach_Zwönitz_Röhrsdorf_CN_166604822_380000_CN_36183042_380000/LConn2
  Markersbach_Zwönitz_Röhrsdorf_CN_166604822_380000_CN_23117075_380000/LConn3 -- T_166604822_380000_Markersbach/LConn3 -- Markersbach_Zwönitz_Röhrsdorf_CN_166604822_380000_CN_36183042_380000/LConn3
  Markersbach_Zwönitz_Röhrsdorf_CN_166604822_380000_CN_23117075_380000/RConn1 -- T_23117075_380000;220000;110000_Umspannwerk_Röhrsdorf/LConn1 -- 574_Remptendorf___Röhrsdorf;_573_Remptendorf___Weida_CN_128277645_380000_CN_23117075_380000/LConn1 -- 572_CN_23117075_380000_CN_157328339_380000/LConn1 -- Schmölln___Dresden_Süd___Röhrsdorf_CN_157807291_380000_CN_23117075_380000/LConn1
  Markersbach_Zwönitz_Röhrsdorf_CN_166604822_380000_CN_23117075_380000/RConn2 -- T_23117075_380000;220000;110000_Umspannwerk_Röhrsdorf/LConn2 -- 574_Remptendorf___Röhrsdorf;_573_Remptendorf___Weida_CN_128277645_380000_CN_23117075_380000/LConn2 -- 572_CN_23117075_380000_CN_157328339_380000/LConn2 -- Schmölln___Dresden_Süd___Röhrsdorf_CN_157807291_380000_CN_23117075_380000/LConn2
  Markersbach_Zwönitz_Röhrsdorf_CN_166604822_380000_CN_23117075_380000/RConn3 -- T_23117075_380000;220000;110000_Umspannwerk_Röhrsdorf/LConn3 -- 574_Remptendorf___Röhrsdorf;_573_Remptendorf___Weida_CN_128277645_380000_CN_23117075_380000/LConn3 -- 572_CN_23117075_380000_CN_157328339_380000/LConn3 -- Schmölln___Dresden_Süd___Röhrsdorf_CN_157807291_380000_CN_23117075_380000/LConn3
  T_36183042_380000;110000_Umspannwerk_Zwönitz/LConn1 -- Markersbach_Zwönitz_Röhrsdorf_CN_166604822_380000_CN_36183042_380000/RConn1
  T_36183042_380000;110000_Umspannwerk_Zwönitz/LConn2 -- Markersbach_Zwönitz_Röhrsdorf_CN_166604822_380000_CN_36183042_380000/RConn2
  T_36183042_380000;110000_Umspannwerk_Zwönitz/LConn3 -- Markersbach_Zwönitz_Röhrsdorf_CN_166604822_380000_CN_36183042_380000/RConn3
  Leitung_2010_CN_113047581_220000_CN-2022229/LConn1 -- T_113047581_380000;220000;110000_Sottrum/RConn1 -- Leitung_2010_CN_113047581_220000_CN_28812249_220000/LConn1 -- Abbenfleth_Sottrum_CN_113047581_220000_CN_24502420_220000/LConn1 -- Abbenfleth_Sottrum_CN_113047581_220000_CN_29344008_220000/LConn1 -- Abbenfleth_Sottrum_CN_113047581_220000_CN_33017336_220000/LConn1 -- Leitung_2144_CN_113047581_220000_CN_229565743_220000/LConn1 -- Leitung_2144_CN_113047581_220000_CN313937042/LConn1 -- L_113047581/LConn1
  Leitung_2010_CN_113047581_220000_CN-2022229/LConn2 -- T_113047581_380000;220000;110000_Sottrum/RConn2 -- Leitung_2010_CN_113047581_220000_CN_28812249_220000/LConn2 -- Abbenfleth_Sottrum_CN_113047581_220000_CN_24502420_220000/LConn2 -- Abbenfleth_Sottrum_CN_113047581_220000_CN_29344008_220000/LConn2 -- Abbenfleth_Sottrum_CN_113047581_220000_CN_33017336_220000/LConn2 -- Leitung_2144_CN_113047581_220000_CN_229565743_220000/LConn2 -- Leitung_2144_CN_113047581_220000_CN313937042/LConn2 -- L_113047581/LConn2
  Leitung_2010_CN_113047581_220000_CN-2022229/LConn3 -- T_113047581_380000;220000;110000_Sottrum/RConn3 -- Leitung_2010_CN_113047581_220000_CN_28812249_220000/LConn3 -- Abbenfleth_Sottrum_CN_113047581_220000_CN_24502420_220000/LConn3 -- Abbenfleth_Sottrum_CN_113047581_220000_CN_29344008_220000/LConn3 -- Abbenfleth_Sottrum_CN_113047581_220000_CN_33017336_220000/LConn3 -- Leitung_2144_CN_113047581_220000_CN_229565743_220000/LConn3 -- Leitung_2144_CN_113047581_220000_CN313937042/LConn3 -- L_113047581/LConn3
  Leitung_2010_CN_113047581_220000_CN-2022229/RConn1 -- G_-2022229_Kraftwerk_Robert_Frank/RConn1 -- Leitung_2008_CN_33042984_220000_CN-2022229/LConn1 -- 2016_CN_23682013_220000_CN-2022229/LConn1 -- Leitung_2008_CN_28921360_220000_CN-2022229/LConn1 -- _CN_27739871_380000_CN-2022229/LConn1
  Leitung_2010_CN_113047581_220000_CN-2022229/RConn2 -- G_-2022229_Kraftwerk_Robert_Frank/RConn2 -- Leitung_2008_CN_33042984_220000_CN-2022229/LConn2 -- 2016_CN_23682013_220000_CN-2022229/LConn2 -- Leitung_2008_CN_28921360_220000_CN-2022229/LConn2 -- _CN_27739871_380000_CN-2022229/LConn2
  Leitung_2010_CN_113047581_220000_CN-2022229/RConn3 -- G_-2022229_Kraftwerk_Robert_Frank/RConn3 -- Leitung_2008_CN_33042984_220000_CN-2022229/LConn3 -- 2016_CN_23682013_220000_CN-2022229/LConn3 -- Leitung_2008_CN_28921360_220000_CN-2022229/LConn3 -- _CN_27739871_380000_CN-2022229/LConn3
  T_28812249_220000;110000_Wechold/LConn1 -- Leitung_2010_CN_113047581_220000_CN_28812249_220000/RConn1
  T_28812249_220000;110000_Wechold/LConn2 -- Leitung_2010_CN_113047581_220000_CN_28812249_220000/RConn2
  T_28812249_220000;110000_Wechold/LConn3 -- Leitung_2010_CN_113047581_220000_CN_28812249_220000/RConn3
  3003_Sottrum___Landsbergen_CN_113047581_380000_CN_27739871_380000/LConn1 -- T_113047581_380000;220000;110000_Sottrum/LConn1 -- 3003_Dollern___Landsbergen_CN_113047581_380000_CN_24502420_380000/LConn1
  3003_Sottrum___Landsbergen_CN_113047581_380000_CN_27739871_380000/LConn2 -- T_113047581_380000;220000;110000_Sottrum/LConn2 -- 3003_Dollern___Landsbergen_CN_113047581_380000_CN_24502420_380000/LConn2
  3003_Sottrum___Landsbergen_CN_113047581_380000_CN_27739871_380000/LConn3 -- T_113047581_380000;220000;110000_Sottrum/LConn3 -- 3003_Dollern___Landsbergen_CN_113047581_380000_CN_24502420_380000/LConn3
  3003_Sottrum___Landsbergen_CN_113047581_380000_CN_27739871_380000/RConn1 -- T_27739871_380000;220000_Landesbergen/LConn1 -- _CN_33411203_380000_CN_27739871_380000/LConn1 -- _CN_27739871_380000_CN-2022229/RConn1 -- Leitung_3011_CN_27739871_380000_CN_24413992_380000/RConn1
  3003_Sottrum___Landsbergen_CN_113047581_380000_CN_27739871_380000/RConn2 -- T_27739871_380000;220000_Landesbergen/LConn2 -- _CN_33411203_380000_CN_27739871_380000/LConn2 -- _CN_27739871_380000_CN-2022229/RConn2 -- Leitung_3011_CN_27739871_380000_CN_24413992_380000/RConn2
  3003_Sottrum___Landsbergen_CN_113047581_380000_CN_27739871_380000/RConn3 -- T_27739871_380000;220000_Landesbergen/LConn3 -- _CN_33411203_380000_CN_27739871_380000/LConn3 -- _CN_27739871_380000_CN-2022229/RConn3 -- Leitung_3011_CN_27739871_380000_CN_24413992_380000/RConn3
  Abbenfleth_Sottrum_CN_113047581_220000_CN_24502420_220000/RConn1 -- T_24502420_380000;220000;110000_Dollern/RConn1 -- L_24502420/LConn1
  Abbenfleth_Sottrum_CN_113047581_220000_CN_24502420_220000/RConn2 -- T_24502420_380000;220000;110000_Dollern/RConn2 -- L_24502420/LConn2
  Abbenfleth_Sottrum_CN_113047581_220000_CN_24502420_220000/RConn3 -- T_24502420_380000;220000;110000_Dollern/RConn3 -- L_24502420/LConn3
  Abbenfleth_Sottrum_CN_113047581_220000_CN_29344008_220000/RConn1 -- T_29344008_220000;110000_Stade/LConn1 -- _CN_29344008_220000_CN_28008024_220000/LConn1 -- _CN_29344008_220000_CN_25306938_220000/LConn1 -- _CN_29344008_220000_CN_151765495_220000/LConn1 -- _CN_29344008_220000_CN_33017336_220000/LConn1
  Abbenfleth_Sottrum_CN_113047581_220000_CN_29344008_220000/RConn2 -- T_29344008_220000;110000_Stade/LConn2 -- _CN_29344008_220000_CN_28008024_220000/LConn2 -- _CN_29344008_220000_CN_25306938_220000/LConn2 -- _CN_29344008_220000_CN_151765495_220000/LConn2 -- _CN_29344008_220000_CN_33017336_220000/LConn2
  Abbenfleth_Sottrum_CN_113047581_220000_CN_29344008_220000/RConn3 -- T_29344008_220000;110000_Stade/LConn3 -- _CN_29344008_220000_CN_28008024_220000/LConn3 -- _CN_29344008_220000_CN_25306938_220000/LConn3 -- _CN_29344008_220000_CN_151765495_220000/LConn3 -- _CN_29344008_220000_CN_33017336_220000/LConn3
  Abbenfleth_Sottrum_CN_113047581_220000_CN_33017336_220000/RConn1 -- T_33017336_220000_Abbenfleth/LConn1 -- _CN_29344008_220000_CN_33017336_220000/RConn1
  Abbenfleth_Sottrum_CN_113047581_220000_CN_33017336_220000/RConn2 -- T_33017336_220000_Abbenfleth/LConn2 -- _CN_29344008_220000_CN_33017336_220000/RConn2
  Abbenfleth_Sottrum_CN_113047581_220000_CN_33017336_220000/RConn3 -- T_33017336_220000_Abbenfleth/LConn3 -- _CN_29344008_220000_CN_33017336_220000/RConn3
  T_229565743_220000;110000_Umspannwerk_Blockland/LConn1 -- Leitung_2144_CN_113047581_220000_CN_229565743_220000/RConn1
  T_229565743_220000;110000_Umspannwerk_Blockland/LConn2 -- Leitung_2144_CN_113047581_220000_CN_229565743_220000/RConn2
  T_229565743_220000;110000_Umspannwerk_Blockland/LConn3 -- Leitung_2144_CN_113047581_220000_CN_229565743_220000/RConn3
  Leitung_2144_CN_113047581_220000_CN313937042/RConn1 -- G_313937042_Kraftwerk_Farge/RConn1 -- _CN_266684854_380000_CN313937042/LConn1 -- 303_CN_44717036_380000_CN313937042/LConn1
  Leitung_2144_CN_113047581_220000_CN313937042/RConn2 -- G_313937042_Kraftwerk_Farge/RConn2 -- _CN_266684854_380000_CN313937042/LConn2 -- 303_CN_44717036_380000_CN313937042/LConn2
  Leitung_2144_CN_113047581_220000_CN313937042/RConn3 -- G_313937042_Kraftwerk_Farge/RConn3 -- _CN_266684854_380000_CN313937042/LConn3 -- 303_CN_44717036_380000_CN313937042/LConn3
  3003_Dollern___Landsbergen_CN_113047581_380000_CN_24502420_380000/RConn1 -- T_24502420_380000;220000;110000_Dollern/LConn1 -- F_CN_24502420_380000_CN_11285720_380000/LConn1 -- 3105_CN_24502420_380000_CN_28502915_380000/LConn1 -- 3105_CN_24502420_380000_CN275650140/LConn1 -- _CN_24502420_380000_CN_31927411_380000/LConn1
  3003_Dollern___Landsbergen_CN_113047581_380000_CN_24502420_380000/RConn2 -- T_24502420_380000;220000;110000_Dollern/LConn2 -- F_CN_24502420_380000_CN_11285720_380000/LConn2 -- 3105_CN_24502420_380000_CN_28502915_380000/LConn2 -- 3105_CN_24502420_380000_CN275650140/LConn2 -- _CN_24502420_380000_CN_31927411_380000/LConn2
  3003_Dollern___Landsbergen_CN_113047581_380000_CN_24502420_380000/RConn3 -- T_24502420_380000;220000;110000_Dollern/LConn3 -- F_CN_24502420_380000_CN_11285720_380000/LConn3 -- 3105_CN_24502420_380000_CN_28502915_380000/LConn3 -- 3105_CN_24502420_380000_CN275650140/LConn3 -- _CN_24502420_380000_CN_31927411_380000/LConn3
  Leupolz___Oberottmarshausen_CN_57727006_380000_CN_77038371_380000/LConn1 -- T_57727006_380000;220000_Schaltanlage_Leupolz/LConn1 -- Vöhringen_Ost;_Füssen_West_CN_57727006_380000_CN_85523877_380000/LConn1 -- Vöhringen_Ost;_Füssen_West_CN_57727006_380000_CN_30613895_380000/LConn1
  Leupolz___Oberottmarshausen_CN_57727006_380000_CN_77038371_380000/LConn2 -- T_57727006_380000;220000_Schaltanlage_Leupolz/LConn2 -- Vöhringen_Ost;_Füssen_West_CN_57727006_380000_CN_85523877_380000/LConn2 -- Vöhringen_Ost;_Füssen_West_CN_57727006_380000_CN_30613895_380000/LConn2
  Leupolz___Oberottmarshausen_CN_57727006_380000_CN_77038371_380000/LConn3 -- T_57727006_380000;220000_Schaltanlage_Leupolz/LConn3 -- Vöhringen_Ost;_Füssen_West_CN_57727006_380000_CN_85523877_380000/LConn3 -- Vöhringen_Ost;_Füssen_West_CN_57727006_380000_CN_30613895_380000/LConn3
  T_77038371_380000;110000_Umspannwerk_Bidingen_Nr__697_S/LConn1 -- Leupolz___Oberottmarshausen_CN_57727006_380000_CN_77038371_380000/RConn1
  T_77038371_380000;110000_Umspannwerk_Bidingen_Nr__697_S/LConn2 -- Leupolz___Oberottmarshausen_CN_57727006_380000_CN_77038371_380000/RConn2
  T_77038371_380000;110000_Umspannwerk_Bidingen_Nr__697_S/LConn3 -- Leupolz___Oberottmarshausen_CN_57727006_380000_CN_77038371_380000/RConn3
  Vöhringen_Ost;_Füssen_West_CN_57727006_220000_CN_25487161_220000/LConn1 -- T_57727006_380000;220000_Schaltanlage_Leupolz/RConn1 -- Vöhringen_Ost;_Füssen_West_CN_57727006_220000_CN_34414970_220000/LConn1 -- Vöhringen_Ost;_Füssen_West_CN_57727006_220000_CN_46766896_220000/LConn1 -- L_57727006/LConn1 -- Vöhringen_Ost;_Füssen_West_CN_57727006_220000_CN_31019937_220000/LConn1 -- Vöhringen_Ost;_Füssen_West_CN_57727006_220000_CN_27200252_220000/LConn1 -- Vöhringen_Ost;_Füssen_West_CN_57727006_220000_CN_30613895_220000/LConn1
  Vöhringen_Ost;_Füssen_West_CN_57727006_220000_CN_25487161_220000/LConn2 -- T_57727006_380000;220000_Schaltanlage_Leupolz/RConn2 -- Vöhringen_Ost;_Füssen_West_CN_57727006_220000_CN_34414970_220000/LConn2 -- Vöhringen_Ost;_Füssen_West_CN_57727006_220000_CN_46766896_220000/LConn2 -- L_57727006/LConn2 -- Vöhringen_Ost;_Füssen_West_CN_57727006_220000_CN_31019937_220000/LConn2 -- Vöhringen_Ost;_Füssen_West_CN_57727006_220000_CN_27200252_220000/LConn2 -- Vöhringen_Ost;_Füssen_West_CN_57727006_220000_CN_30613895_220000/LConn2
  Vöhringen_Ost;_Füssen_West_CN_57727006_220000_CN_25487161_220000/LConn3 -- T_57727006_380000;220000_Schaltanlage_Leupolz/RConn3 -- Vöhringen_Ost;_Füssen_West_CN_57727006_220000_CN_34414970_220000/LConn3 -- Vöhringen_Ost;_Füssen_West_CN_57727006_220000_CN_46766896_220000/LConn3 -- L_57727006/LConn3 -- Vöhringen_Ost;_Füssen_West_CN_57727006_220000_CN_31019937_220000/LConn3 -- Vöhringen_Ost;_Füssen_West_CN_57727006_220000_CN_27200252_220000/LConn3 -- Vöhringen_Ost;_Füssen_West_CN_57727006_220000_CN_30613895_220000/LConn3
  T_25487161_220000;110000_Umspannwerk_Memmingen/LConn1 -- Vöhringen_Ost;_Füssen_West_CN_57727006_220000_CN_25487161_220000/RConn1
  T_25487161_220000;110000_Umspannwerk_Memmingen/LConn2 -- Vöhringen_Ost;_Füssen_West_CN_57727006_220000_CN_25487161_220000/RConn2
  T_25487161_220000;110000_Umspannwerk_Memmingen/LConn3 -- Vöhringen_Ost;_Füssen_West_CN_57727006_220000_CN_25487161_220000/RConn3
  Vöhringen_Ost;_Füssen_West_CN_57727006_220000_CN_31019937_220000/RConn1 -- T_31019937_380000;220000;110000_Vöhringen_LEW/RConn1 -- Iller_Ltg__CN_31019937_220000_CN_41389594_220000/LConn1 -- L_31019937/LConn1 -- _CN_30613895_220000_CN_31019937_220000/LConn1
  Vöhringen_Ost;_Füssen_West_CN_57727006_220000_CN_31019937_220000/RConn2 -- T_31019937_380000;220000;110000_Vöhringen_LEW/RConn2 -- Iller_Ltg__CN_31019937_220000_CN_41389594_220000/LConn2 -- L_31019937/LConn2 -- _CN_30613895_220000_CN_31019937_220000/LConn2
  Vöhringen_Ost;_Füssen_West_CN_57727006_220000_CN_31019937_220000/RConn3 -- T_31019937_380000;220000;110000_Vöhringen_LEW/RConn3 -- Iller_Ltg__CN_31019937_220000_CN_41389594_220000/LConn3 -- L_31019937/LConn3 -- _CN_30613895_220000_CN_31019937_220000/LConn3
  Vöhringen_Ost;_Füssen_West_CN_57727006_380000_CN_85523877_380000/RConn1 -- T_85523877_380000_Vöhringen_Amprion/LConn1 -- _CN_85523877_380000_CN_41389594_380000/LConn1 -- Meitingen_Nord;_Süd_CN_24652261_380000_CN_85523877_380000/LConn1 -- _CN_31019937_380000_CN_85523877_380000/LConn1
  Vöhringen_Ost;_Füssen_West_CN_57727006_380000_CN_85523877_380000/RConn2 -- T_85523877_380000_Vöhringen_Amprion/LConn2 -- _CN_85523877_380000_CN_41389594_380000/LConn2 -- Meitingen_Nord;_Süd_CN_24652261_380000_CN_85523877_380000/LConn2 -- _CN_31019937_380000_CN_85523877_380000/LConn2
  Vöhringen_Ost;_Füssen_West_CN_57727006_380000_CN_85523877_380000/RConn3 -- T_85523877_380000_Vöhringen_Amprion/LConn3 -- _CN_85523877_380000_CN_41389594_380000/LConn3 -- Meitingen_Nord;_Süd_CN_24652261_380000_CN_85523877_380000/LConn3 -- _CN_31019937_380000_CN_85523877_380000/LConn3
  T_27200252_220000;110000_Umspannstation_Irsingen/LConn1 -- Vöhringen_Ost;_Füssen_West_CN_57727006_220000_CN_27200252_220000/RConn1
  T_27200252_220000;110000_Umspannstation_Irsingen/LConn2 -- Vöhringen_Ost;_Füssen_West_CN_57727006_220000_CN_27200252_220000/RConn2
  T_27200252_220000;110000_Umspannstation_Irsingen/LConn3 -- Vöhringen_Ost;_Füssen_West_CN_57727006_220000_CN_27200252_220000/RConn3
  Vöhringen_Ost;_Füssen_West_CN_57727006_220000_CN_30613895_220000/RConn1 -- T_30613895_380000;220000;110000_Umspannwerk_Oberottmarshausen/RConn1 -- _CN_30613895_220000_CN_31019937_220000/RConn1 -- L_30613895/LConn1
  Vöhringen_Ost;_Füssen_West_CN_57727006_220000_CN_30613895_220000/RConn2 -- T_30613895_380000;220000;110000_Umspannwerk_Oberottmarshausen/RConn2 -- _CN_30613895_220000_CN_31019937_220000/RConn2 -- L_30613895/LConn2
  Vöhringen_Ost;_Füssen_West_CN_57727006_220000_CN_30613895_220000/RConn3 -- T_30613895_380000;220000;110000_Umspannwerk_Oberottmarshausen/RConn3 -- _CN_30613895_220000_CN_31019937_220000/RConn3 -- L_30613895/LConn3
  Vöhringen_Ost;_Füssen_West_CN_57727006_380000_CN_30613895_380000/RConn1 -- T_30613895_380000;220000;110000_Umspannwerk_Oberottmarshausen/LConn1 -- _CN_30613895_380000_CN_53378027_380000/LConn1 -- _CN_30613895_380000_CN_24652261_380000/LConn1
  Vöhringen_Ost;_Füssen_West_CN_57727006_380000_CN_30613895_380000/RConn2 -- T_30613895_380000;220000;110000_Umspannwerk_Oberottmarshausen/LConn2 -- _CN_30613895_380000_CN_53378027_380000/LConn2 -- _CN_30613895_380000_CN_24652261_380000/LConn2
  Vöhringen_Ost;_Füssen_West_CN_57727006_380000_CN_30613895_380000/RConn3 -- T_30613895_380000;220000;110000_Umspannwerk_Oberottmarshausen/LConn3 -- _CN_30613895_380000_CN_53378027_380000/LConn3 -- _CN_30613895_380000_CN_24652261_380000/LConn3
  T_34414970_220000;110000_Umspannwerk_Rauhenzell/LConn1 -- Vöhringen_Ost;_Füssen_West_CN_57727006_220000_CN_34414970_220000/RConn1
  T_34414970_220000;110000_Umspannwerk_Rauhenzell/LConn2 -- Vöhringen_Ost;_Füssen_West_CN_57727006_220000_CN_34414970_220000/RConn2
  T_34414970_220000;110000_Umspannwerk_Rauhenzell/LConn3 -- Vöhringen_Ost;_Füssen_West_CN_57727006_220000_CN_34414970_220000/RConn3
  Vöhringen_Ost;_Füssen_West_CN_57727006_220000_CN_46766896_220000/RConn1 -- T_46766896_220000_Schaltwerk_Kempten/LConn1 -- _CN_46766896_220000_CN_90807341_220000/LConn1
  Vöhringen_Ost;_Füssen_West_CN_57727006_220000_CN_46766896_220000/RConn2 -- T_46766896_220000_Schaltwerk_Kempten/LConn2 -- _CN_46766896_220000_CN_90807341_220000/LConn2
  Vöhringen_Ost;_Füssen_West_CN_57727006_220000_CN_46766896_220000/RConn3 -- T_46766896_220000_Schaltwerk_Kempten/LConn3 -- _CN_46766896_220000_CN_90807341_220000/LConn3
  220_kV_Rheinau_Ost|West_CN_147521567_220000_CN_149987048_220000/LConn1 -- T_147521567_220000;110000_Umspannanlage_Pfungstadt/LConn1 -- 220_kV_Rheinau_Ost|West_CN_147521567_220000_CN_152022992_220000/LConn1 -- 220_kV_Rheinau_Ost|West_CN_147521567_220000_CN_152973139_220000/RConn1
  220_kV_Rheinau_Ost|West_CN_147521567_220000_CN_149987048_220000/LConn2 -- T_147521567_220000;110000_Umspannanlage_Pfungstadt/LConn2 -- 220_kV_Rheinau_Ost|West_CN_147521567_220000_CN_152022992_220000/LConn2 -- 220_kV_Rheinau_Ost|West_CN_147521567_220000_CN_152973139_220000/RConn2
  220_kV_Rheinau_Ost|West_CN_147521567_220000_CN_149987048_220000/LConn3 -- T_147521567_220000;110000_Umspannanlage_Pfungstadt/LConn3 -- 220_kV_Rheinau_Ost|West_CN_147521567_220000_CN_152022992_220000/LConn3 -- 220_kV_Rheinau_Ost|West_CN_147521567_220000_CN_152973139_220000/RConn3
  220_kV_Rheinau_Ost|West_CN_147521567_220000_CN_149987048_220000/RConn1 -- T_149987048_380000;220000_Station_Bürstadt/RConn1 -- 220_kV_Kondelwald;_220kV_Wengerohr_CN_66764943_220000_CN_149987048_220000/LConn1 -- 220_kV_Anilin_1A|2B_CN_152924508_220000_CN_149987048_220000/LConn1 -- L_149987048/LConn1
  220_kV_Rheinau_Ost|West_CN_147521567_220000_CN_149987048_220000/RConn2 -- T_149987048_380000;220000_Station_Bürstadt/RConn2 -- 220_kV_Kondelwald;_220kV_Wengerohr_CN_66764943_220000_CN_149987048_220000/LConn2 -- 220_kV_Anilin_1A|2B_CN_152924508_220000_CN_149987048_220000/LConn2 -- L_149987048/LConn2
  220_kV_Rheinau_Ost|West_CN_147521567_220000_CN_149987048_220000/RConn3 -- T_149987048_380000;220000_Station_Bürstadt/RConn3 -- 220_kV_Kondelwald;_220kV_Wengerohr_CN_66764943_220000_CN_149987048_220000/LConn3 -- 220_kV_Anilin_1A|2B_CN_152924508_220000_CN_149987048_220000/LConn3 -- L_149987048/LConn3
  220_kV_Rheinau_Ost|West_CN_147521567_220000_CN_152022992_220000/RConn1 -- T_152022992_220000;110000_Niederhausen/LConn1 -- _CN_152107815_220000_CN_152022992_220000/LConn1
  220_kV_Rheinau_Ost|West_CN_147521567_220000_CN_152022992_220000/RConn2 -- T_152022992_220000;110000_Niederhausen/LConn2 -- _CN_152107815_220000_CN_152022992_220000/LConn2
  220_kV_Rheinau_Ost|West_CN_147521567_220000_CN_152022992_220000/RConn3 -- T_152022992_220000;110000_Niederhausen/LConn3 -- _CN_152107815_220000_CN_152022992_220000/LConn3
  304_CN_177829920_380000_CN_23837631_380000/LConn1 -- T_177829920_380000;150000;110000_Diele/LConn1 -- 305_CN_177829920_380000_CN_32042992_380000/LConn1
  304_CN_177829920_380000_CN_23837631_380000/LConn2 -- T_177829920_380000;150000;110000_Diele/LConn2 -- 305_CN_177829920_380000_CN_32042992_380000/LConn2
  304_CN_177829920_380000_CN_23837631_380000/LConn3 -- T_177829920_380000;150000;110000_Diele/LConn3 -- 305_CN_177829920_380000_CN_32042992_380000/LConn3
  304_CN_177829920_380000_CN_23837631_380000/RConn1 -- T_23837631_380000;220000;110000_Conneforde/LConn1 -- 302_CN_23837631_380000_CN_32076853_380000/LConn1
  304_CN_177829920_380000_CN_23837631_380000/RConn2 -- T_23837631_380000;220000;110000_Conneforde/LConn2 -- 302_CN_23837631_380000_CN_32076853_380000/LConn2
  304_CN_177829920_380000_CN_23837631_380000/RConn3 -- T_23837631_380000;220000;110000_Conneforde/LConn3 -- 302_CN_23837631_380000_CN_32076853_380000/LConn3
  305_CN_177829920_380000_CN_32042992_380000/RConn1 -- T_32042992_380000_Umspannwerk_Rhede/LConn1 -- _CN_29077623_380000_CN_32042992_380000/LConn1
  305_CN_177829920_380000_CN_32042992_380000/RConn2 -- T_32042992_380000_Umspannwerk_Rhede/LConn2 -- _CN_29077623_380000_CN_32042992_380000/LConn2
  305_CN_177829920_380000_CN_32042992_380000/RConn3 -- T_32042992_380000_Umspannwerk_Rhede/LConn3 -- _CN_29077623_380000_CN_32042992_380000/LConn3
  Anlage_4508_CN_25786404_220000_CN_25306752_220000/RConn1 -- T_25306752_380000;220000;110000_Umspannwerk_Herbertingen/RConn1 -- Dellmensingen___Obermooweiler;Dellmensingen_Ost_CN_41389594_220000_CN_25306752_220000/LConn1 -- L_25306752/LConn1
  Anlage_4508_CN_25786404_220000_CN_25306752_220000/RConn2 -- T_25306752_380000;220000;110000_Umspannwerk_Herbertingen/RConn2 -- Dellmensingen___Obermooweiler;Dellmensingen_Ost_CN_41389594_220000_CN_25306752_220000/LConn2 -- L_25306752/LConn2
  Anlage_4508_CN_25786404_220000_CN_25306752_220000/RConn3 -- T_25306752_380000;220000;110000_Umspannwerk_Herbertingen/RConn3 -- Dellmensingen___Obermooweiler;Dellmensingen_Ost_CN_41389594_220000_CN_25306752_220000/LConn3 -- L_25306752/LConn3
  _CN_25786404_220000_CN_25802269_220000/RConn1 -- T_25802269_380000;220000;110000_Umspannstation_Hoheneck_Amprion/RConn1 -- L_25802269/LConn1
  _CN_25786404_220000_CN_25802269_220000/RConn2 -- T_25802269_380000;220000;110000_Umspannstation_Hoheneck_Amprion/RConn2 -- L_25802269/LConn2
  _CN_25786404_220000_CN_25802269_220000/RConn3 -- T_25802269_380000;220000;110000_Umspannstation_Hoheneck_Amprion/RConn3 -- L_25802269/LConn3
  T_97825259_220000;110000_Marbach/LConn1 -- Anlage_322_CN_25786404_220000_CN_97825259_220000/RConn1
  T_97825259_220000;110000_Marbach/LConn2 -- Anlage_322_CN_25786404_220000_CN_97825259_220000/RConn2
  T_97825259_220000;110000_Marbach/LConn3 -- Anlage_322_CN_25786404_220000_CN_97825259_220000/RConn3
  T_32205824_220000;110000_Umspannwerk_Winnenden/LConn1 -- Anlage_322_CN_25786404_220000_CN_32205824_220000/RConn1
  T_32205824_220000;110000_Umspannwerk_Winnenden/LConn2 -- Anlage_322_CN_25786404_220000_CN_32205824_220000/RConn2
  T_32205824_220000;110000_Umspannwerk_Winnenden/LConn3 -- Anlage_322_CN_25786404_220000_CN_32205824_220000/RConn3
  Anlage_322_CN_25786404_220000_CN_26260052_220000/RConn1 -- T_26260052_380000;220000;110000_EnBW_Umspannwerk_Wendlingen/RConn1 -- L_26260052/LConn1
  Anlage_322_CN_25786404_220000_CN_26260052_220000/RConn2 -- T_26260052_380000;220000;110000_EnBW_Umspannwerk_Wendlingen/RConn2 -- L_26260052/LConn2
  Anlage_322_CN_25786404_220000_CN_26260052_220000/RConn3 -- T_26260052_380000;220000;110000_EnBW_Umspannwerk_Wendlingen/RConn3 -- L_26260052/LConn3
  Dellmensingen___Niederstotzingen_CN_31105067_380000_CN_38325076_380000/LConn1 -- T_31105067_380000;110000_Umspannwerk_Niederstotzingen/LConn1 -- Dellmensingen___Niederstotzingen_CN_31105067_380000_CN_42050342_380000/LConn1 -- Dellmensingen___Niederstotzingen_CN_31105067_380000_CN_41389594_380000/LConn1
  Dellmensingen___Niederstotzingen_CN_31105067_380000_CN_38325076_380000/LConn2 -- T_31105067_380000;110000_Umspannwerk_Niederstotzingen/LConn2 -- Dellmensingen___Niederstotzingen_CN_31105067_380000_CN_42050342_380000/LConn2 -- Dellmensingen___Niederstotzingen_CN_31105067_380000_CN_41389594_380000/LConn2
  Dellmensingen___Niederstotzingen_CN_31105067_380000_CN_38325076_380000/LConn3 -- T_31105067_380000;110000_Umspannwerk_Niederstotzingen/LConn3 -- Dellmensingen___Niederstotzingen_CN_31105067_380000_CN_42050342_380000/LConn3 -- Dellmensingen___Niederstotzingen_CN_31105067_380000_CN_41389594_380000/LConn3
  T_38325076_380000;110000_Umspannwerk_Rotensohl/LConn1 -- Dellmensingen___Niederstotzingen_CN_31105067_380000_CN_38325076_380000/RConn1
  T_38325076_380000;110000_Umspannwerk_Rotensohl/LConn2 -- Dellmensingen___Niederstotzingen_CN_31105067_380000_CN_38325076_380000/RConn2
  T_38325076_380000;110000_Umspannwerk_Rotensohl/LConn3 -- Dellmensingen___Niederstotzingen_CN_31105067_380000_CN_38325076_380000/RConn3
  Dellmensingen___Niederstotzingen_CN_31105067_380000_CN_42050342_380000/RConn1 -- T_42050342_380000;220000;110000_Umspannwerk_Goldshöfe/LConn1 -- Goldshöfe___Kupferzell_CN_42050342_380000_CN_143854536_380000/LConn1
  Dellmensingen___Niederstotzingen_CN_31105067_380000_CN_42050342_380000/RConn2 -- T_42050342_380000;220000;110000_Umspannwerk_Goldshöfe/LConn2 -- Goldshöfe___Kupferzell_CN_42050342_380000_CN_143854536_380000/LConn2
  Dellmensingen___Niederstotzingen_CN_31105067_380000_CN_42050342_380000/RConn3 -- T_42050342_380000;220000;110000_Umspannwerk_Goldshöfe/LConn3 -- Goldshöfe___Kupferzell_CN_42050342_380000_CN_143854536_380000/LConn3
  Dellmensingen___Niederstotzingen_CN_31105067_380000_CN_41389594_380000/RConn1 -- T_41389594_380000;220000;110000_Umspannwerk_Dellmensingen/LConn1 -- 380_kV_CN_26260052_380000_CN_41389594_380000/LConn1 -- _CN_85523877_380000_CN_41389594_380000/RConn1 -- Dellmensingen___Obermooweiler;Dellmensingen_Ost_CN_41389594_380000_CN_31131320_380000/LConn1
  Dellmensingen___Niederstotzingen_CN_31105067_380000_CN_41389594_380000/RConn2 -- T_41389594_380000;220000;110000_Umspannwerk_Dellmensingen/LConn2 -- 380_kV_CN_26260052_380000_CN_41389594_380000/LConn2 -- _CN_85523877_380000_CN_41389594_380000/RConn2 -- Dellmensingen___Obermooweiler;Dellmensingen_Ost_CN_41389594_380000_CN_31131320_380000/LConn2
